simulink library "GTPR_Library"  (R2021a)
settings: Solver=VariableStepAuto  StartTime=0.0  StopTime=10.0  RelTol=1e-3
values from neighbouring files (symbols this model uses):
  aA = 0.5    [SimMechanics_GTPR_OpenLoop_CircularMotion_VS_ClosedLoop.m]
  aB = 0.5    [SimMechanics_GTPR_OpenLoop_CircularMotion_VS_ClosedLoop.m]
  aC = 0.5    [SimMechanics_GTPR_OpenLoop_CircularMotion_VS_ClosedLoop.m]
  alphaAB = deg2rad(120)    [SimMechanics_GTPR_OpenLoop_CircularMotion_VS_ClosedLoop.m]
  alphaAC = deg2rad(240)    [SimMechanics_GTPR_OpenLoop_CircularMotion_VS_ClosedLoop.m]
  eA = 0.28    [SimMechanics_GTPR_OpenLoop_CircularMotion_VS_ClosedLoop.m]
  eB = 0.28    [SimMechanics_GTPR_OpenLoop_CircularMotion_VS_ClosedLoop.m]
  eC = 0.28    [SimMechanics_GTPR_OpenLoop_CircularMotion_VS_ClosedLoop.m]
  g = -9.81    [SimMechanics_GTPR_OpenLoop_CircularMotion_VS_ClosedLoop.m]
  ILA = zeros(3)    [SimMechanics_GTPR_OpenLoop_CircularMotion_VS_ClosedLoop.m]
  IlA = zeros(3)    [SimMechanics_GTPR_OpenLoop_CircularMotion_VS_ClosedLoop.m]
  ILB = zeros(3)    [SimMechanics_GTPR_OpenLoop_CircularMotion_VS_ClosedLoop.m]
  IlB = zeros(3)    [SimMechanics_GTPR_OpenLoop_CircularMotion_VS_ClosedLoop.m]
  ILC = zeros(3)    [SimMechanics_GTPR_OpenLoop_CircularMotion_VS_ClosedLoop.m]
  IlC = zeros(3)    [SimMechanics_GTPR_OpenLoop_CircularMotion_VS_ClosedLoop.m]
  LA = 0.57    [SimMechanics_GTPR_OpenLoop_CircularMotion_VS_ClosedLoop.m]
  lA = 0.9    [SimMechanics_GTPR_OpenLoop_CircularMotion_VS_ClosedLoop.m]
  LB = 0.57    [SimMechanics_GTPR_OpenLoop_CircularMotion_VS_ClosedLoop.m]
  lB = 0.9    [SimMechanics_GTPR_OpenLoop_CircularMotion_VS_ClosedLoop.m]
  LC = 0.57    [SimMechanics_GTPR_OpenLoop_CircularMotion_VS_ClosedLoop.m]
  lC = 0.9    [SimMechanics_GTPR_OpenLoop_CircularMotion_VS_ClosedLoop.m]
  m_unaccounted = 1e-16    [SimMechanics_GTPR_OpenLoop_CircularMotion_VS_ClosedLoop.m]
  mLA = density_upperArm*VLA    (= 1.4415197891)    [SimMechanics_GTPR_OpenLoop_CircularMotion_VS_ClosedLoop.m]
  mlA = density_LowerArm*VlA    (= 0.190851753706)    [SimMechanics_GTPR_OpenLoop_CircularMotion_VS_ClosedLoop.m]
  mLB = density_upperArm*VLB    (= 1.4415197891)    [SimMechanics_GTPR_OpenLoop_CircularMotion_VS_ClosedLoop.m]
  mlB = density_LowerArm*VlB    (= 0.190851753706)    [SimMechanics_GTPR_OpenLoop_CircularMotion_VS_ClosedLoop.m]
  mLC = density_upperArm*VLC    (= 1.4415197891)    [SimMechanics_GTPR_OpenLoop_CircularMotion_VS_ClosedLoop.m]
  mlC = density_LowerArm*VlC    (= 0.190851753706)    [SimMechanics_GTPR_OpenLoop_CircularMotion_VS_ClosedLoop.m]
  mTCP = density_workTriangle * VTCP    [SimMechanics_GTPR_OpenLoop_CircularMotion_VS_ClosedLoop.m]
undefined symbols (not defined in the file or in its folder): dq1, dq2, dq3, q1, q2, q3, X, Y, Z
libraries: sm_lib x83, $bdroot x31, nesl_utility x24
(part 6 of 8)

== matlab function GTPR_Library/Dynamics/DynamicEquations/Dynamic Eqs ==
  data: Mxyz output; Mddq output; aA input size=1; aB input size=1; aC input; alphaAB input size=1; alphaAC input size=1; LA input size=1; LB input size=1; LC input size=1; lA input size=1; lB input size=1; lC input size=1; eA input size=1; eB input size=1; eC input size=1; q input size=[3 1]; dq input size=[3 1]; ddq input size=[3 1]; TCP input size=[3 1]; ILA input size=[3 3]; ILB input size=[3 3]; ILC input size=[3 3]; IlA input size=[3 3]; IlB input size=[3 3]; IlC input size=[3 3]; a input size=[3 1]; g input size=1; mLA input size=1; mLB input size=1; mLC input size=1; mlA input size=1; mlB input size=1; mlC input size=1; mTCP input size=1; dGammasdq output; Fext input size=[3 1]; lambda output; Mtimesddq output; M output; f output; tau output; v input; J11 input; J12 input; J13 input; J21 input; J22 input; J23 input; J31 input; J32 input; J33 input
function [Mxyz, Mddq, dGammasdq, lambda, Mtimesddq, M, f, tau] = Dynamics(aA, aB, aC, alphaAB, alphaAC, LA, LB, LC, lA, lB, lC, eA, eB, eC, q, dq, ddq,TCP, ILA, ILB, ILC, IlA, IlB, IlC, a, g, mLA, mLB, mLC, mlA, mlB, mlC, mTCP, Fext, v, J11, J12, J13, J21, J22, J23, J31, J32, J33) 

alphaAA = 0;

q1 = q(1);
q2 = q(2);
q3 = q(3);

dq1 = dq(1);
dq2 = dq(2);
dq3 = dq(3);

ddq1 = ddq(1);
ddq2 = ddq(2);
ddq3 = ddq(3);

x = TCP(1);
y = TCP(2);
z = TCP(3);

dx = v(1);
dy = v(2);
dz = v(3);

ddx = a(1);
ddy = a(2);
ddz = a(3);

ILAxx = ILA(1,1);
ILAxy = ILA(1,2);
% ILAxz = ILA(1,3);
ILAyy = ILA(2,2);
% ILAyz = ILA(2,3);
% ILAzz = ILA(3,3);

ILBxx = ILB(1,1);
ILBxy = ILB(1,2);
% ILBxz = ILB(1,3);
ILByy = ILB(2,2);
% ILByz = ILB(2,3);
% ILBzz = ILB(3,3);

ILCxx = ILC(1,1);
ILCxy = ILC(1,2);
% ILCxz = ILC(1,3);
ILCyy = ILC(2,2);
% ILCyz = ILC(2,3);
% ILCzz = ILC(3,3);

IlAxx = IlA(1,1);
IlAxy = IlA(1,2);
IlAxz = IlA(1,3);
IlAyy = IlA(2,2);
IlAyz = IlA(2,3);
IlAzz = IlA(3,3);

IlBxx = IlB(1,1);
IlBxy = IlB(1,2);
IlBxz = IlB(1,3);
IlByy = IlB(2,2);
IlByz = IlB(2,3);
IlBzz = IlB(3,3);

IlCxx = IlC(1,1);
IlCxy = IlC(1,2);
IlCxz = IlC(1,3);
IlCyy = IlC(2,2);
IlCyz = IlC(2,3);
IlCzz = IlC(3,3);

J = [J11, J12, J13; J21, J22, J23; J31, J32, J33];

dGammasdxyz = reshape([x.*2.0+aA.*sin(alphaAA).*2.0-eA.*sin(alphaAA).*2.0+LA.*cos(q1).*sin(alphaAA).*2.0,y.*2.0+aA.*cos(alphaAA).*2.0-eA.*cos(alphaAA).*2.0+LA.*cos(alphaAA).*cos(q1).*2.0,z.*2.0+LA.*sin(q1).*2.0,x.*2.0+aB.*sin(alphaAB).*2.0-eB.*sin(alphaAB).*2.0+LB.*cos(q2).*sin(alphaAB).*2.0,y.*2.0+aB.*cos(alphaAB).*2.0-eB.*cos(alphaAB).*2.0+LB.*cos(alphaAB).*cos(q2).*2.0,z.*2.0+LB.*sin(q2).*2.0,x.*2.0+aC.*sin(alphaAC).*2.0-eC.*sin(alphaAC).*2.0+LC.*cos(q3).*sin(alphaAC).*2.0,y.*2.0+aC.*cos(alphaAC).*2.0-eC.*cos(alphaAC).*2.0+LC.*cos(alphaAC).*cos(q3).*2.0,z.*2.0+LC.*sin(q3).*2.0],[3,3]);
Mxyz = [(mlA.*(ddx./2.0+(LA.*dq1.^2.*cos(q1).*cos(alphaAA-pi./2.0))./2.0+(LA.*ddq1.*sin(q1).*cos(alphaAA-pi./2.0))./2.0))./2.0+mlA.*(ddx./4.0+(LA.*dq1.^2.*cos(q1).*cos(alphaAA-pi./2.0))./4.0+(LA.*ddq1.*sin(q1).*cos(alphaAA-pi./2.0))./4.0)+(mlB.*(ddx./2.0+(LB.*dq2.^2.*cos(q2).*cos(alphaAB-pi./2.0))./2.0+(LB.*ddq2.*sin(q2).*cos(alphaAB-pi./2.0))./2.0))./2.0+mlB.*(ddx./4.0+(LB.*dq2.^2.*cos(q2).*cos(alphaAB-pi./2.0))./4.0+(LB.*ddq2.*sin(q2).*cos(alphaAB-pi./2.0))./4.0)+(mlC.*(ddx./2.0+(LC.*dq3.^2.*cos(q3).*cos(alphaAC-pi./2.0))./2.0+(LC.*ddq3.*sin(q3).*cos(alphaAC-pi./2.0))./2.0))./2.0+mlC.*(ddx./4.0+(LC.*dq3.^2.*cos(q3).*cos(alphaAC-pi./2.0))./4.0+(LC.*ddq3.*sin(q3).*cos(alphaAC-pi./2.0))./4.0)+ddx.*mTCP+(((IlAxz.*1.0./lA.^2.*(y+aA.*cos(alphaAA)-eA.*cos(alphaAA)+LA.*cos(alphaAA).*cos(q1)))./2.0-(IlAxy.*1.0./lA.^2.*(z+LA.*sin(q1)))./2.0).*(((dz+LA.*dq1.*cos(q1)).*(dy+LA.*dq1.*sin(alphaAA-pi./2.0).*sin(q1)))./lA-((dy-LA.*dq1.*cos(alphaAA).*sin(q1)).*(dz+LA.*dq1.*sin(pi./2.0).*cos(q1)))./lA+((z+LA.*sin(q1)).*(ddy+LA.*dq1.^2.*sin(alphaAA-pi./2.0).*cos(q1)+LA.*ddq1.*sin(alphaAA-pi./2.0).*sin(q1)))./lA-((ddz+LA.*ddq1.*sin(pi./2.0).*cos(q1)-LA.*dq1.^2.*sin(pi./2.0).*sin(q1)).*(y+aA.*cos(alphaAA)-eA.*cos(alphaAA)+LA.*cos(alphaAA).*cos(q1)))./lA).*2.0)./lA+(((IlBxz.*1.0./lB.^2.*(y+aB.*cos(alphaAB)-eB.*cos(alphaAB)+LB.*cos(alphaAB).*cos(q2)))./2.0-(IlBxy.*1.0./lB.^2.*(z+LB.*sin(q2)))./2.0).*(((dz+LB.*dq2.*cos(q2)).*(dy+LB.*dq2.*sin(alphaAB-pi./2.0).*sin(q2)))./lB-((dy-LB.*dq2.*cos(alphaAB).*sin(q2)).*(dz+LB.*dq2.*sin(pi./2.0).*cos(q2)))./lB+((z+LB.*sin(q2)).*(ddy+LB.*dq2.^2.*sin(alphaAB-pi./2.0).*cos(q2)+LB.*ddq2.*sin(alphaAB-pi./2.0).*sin(q2)))./lB-((ddz+LB.*ddq2.*sin(pi./2.0).*cos(q2)-LB.*dq2.^2.*sin(pi./2.0).*sin(q2)).*(y+aB.*cos(alphaAB)-eB.*cos(alphaAB)+LB.*cos(alphaAB).*cos(q2)))./lB).*2.0)./lB+(((IlCxz.*1.0./lC.^2.*(y+aC.*cos(alphaAC)-eC.*cos(alphaAC)+LC.*cos(alphaAC).*cos(q3)))./2.0-(IlCxy.*1.0./lC.^2.*(z+LC.*sin(q3)))./2.0).*(((dz+LC.*dq3.*cos(q3)).*(dy+LC.*dq3.*sin(alphaAC-pi./2.0).*sin(q3)))./lC-((dy-LC.*dq3.*cos(alphaAC).*sin(q3)).*(dz+LC.*dq3.*sin(pi./2.0).*cos(q3)))./lC+((z+LC.*sin(q3)).*(ddy+LC.*dq3.^2.*sin(alphaAC-pi./2.0).*cos(q3)+LC.*ddq3.*sin(alphaAC-pi./2.0).*sin(q3)))./lC-((ddz+LC.*ddq3.*sin(pi./2.0).*cos(q3)-LC.*dq3.^2.*sin(pi./2.0).*sin(q3)).*(y+aC.*cos(alphaAC)-eC.*cos(alphaAC)+LC.*cos(alphaAC).*cos(q3)))./lC).*2.0)./lC-(((IlAxz.*1.0./lA.^2.*(dy+LA.*dq1.*sin(alphaAA-pi./2.0).*sin(q1)))./2.0-(IlAxy.*1.0./lA.^2.*(dz+LA.*dq1.*sin(pi./2.0).*cos(q1)))./2.0).*(((dz+LA.*dq1.*sin(pi./2.0).*cos(q1)).*(y+aA.*cos(alphaAA)-eA.*cos(alphaAA)+LA.*cos(alphaAA).*cos(q1)))./lA-((z+LA.*sin(q1)).*(dy+LA.*dq1.*sin(alphaAA-pi./2.0).*sin(q1)))./lA).*2.0)./lA-(((IlBxz.*1.0./lB.^2.*(dy+LB.*dq2.*sin(alphaAB-pi./2.0).*sin(q2)))./2.0-(IlBxy.*1.0./lB.^2.*(dz+LB.*dq2.*sin(pi./2.0).*cos(q2)))./2.0).*(((dz+LB.*dq2.*sin(pi./2.0).*cos(q2)).*(y+aB.*cos(alphaAB)-eB.*cos(alphaAB)+LB.*cos(alphaAB).*cos(q2)))./lB-((z+LB.*sin(q2)).*(dy+LB.*dq2.*sin(alphaAB-pi./2.0).*sin(q2)))./lB).*2.0)./lB-(((IlCxz.*1.0./lC.^2.*(dy+LC.*dq3.*sin(alphaAC-pi./2.0).*sin(q3)))./2.0-(IlCxy.*1.0./lC.^2.*(dz+LC.*dq3.*sin(pi./2.0).*cos(q3)))./2.0).*(((dz+LC.*dq3.*sin(pi./2.0).*cos(q3)).*(y+aC.*cos(alphaAC)-eC.*cos(alphaAC)+LC.*cos(alphaAC).*cos(q3)))./lC-((z+LC.*sin(q3)).*(dy+LC.*dq3.*sin(alphaAC-pi./2.0).*sin(q3)))./lC).*2.0)./lC-1.0./lA.^2.*(dy-LA.*dq1.*cos(alphaAA).*sin(q1)).*((IlAzz.*(((dx-LA.*dq1.*sin(q1).*cos(alphaAA-pi./2.0)).*(y+aA.*cos(alphaAA)-eA.*cos(alphaAA)+LA.*cos(alphaAA).*cos(q1)))./lA-((dy+LA.*dq1.*sin(alphaAA-pi./2.0).*sin(q1)).*(x+aA.*sin(alphaAA)-eA.*sin(alphaAA)+LA.*cos(q1).*sin(alphaAA)))./lA).*(-1.0./2.0))./lA+(IlAxz.*(((dz+LA.*dq1.*sin(pi./2.0).*cos(q1)).*(y+aA.*cos(alphaAA)-eA.*cos(alphaAA)+LA.*cos(alphaAA).*cos(q1)))./lA-((z+LA.*sin(q1)).*(dy+LA.*dq1.*sin(alphaAA-pi./2.0).*sin(q1)))./lA))./(lA.*2.0)+(IlAyz.*(((z+LA.*sin(q1)).*(dx-LA.*dq1.*sin(q1).*cos(alphaAA-pi./2.0)))./lA-((dz+LA.*dq1.*sin(pi./2.0).*cos(q1)).*(x+aA.*sin(alphaAA)-eA.*sin(alphaAA)+LA.*cos(q1).*sin(alphaAA)))./lA))./(lA.*2.0)).*2.0-1.0./lB.^2.*(dy-LB.*dq2.*cos(alphaAB).*sin(q2)).*((IlBzz.*(((dx-LB.*dq2.*sin(q2).*cos(alphaAB-pi./2.0)).*(y+aB.*cos(alphaAB)-eB.*cos(alphaAB)+LB.*cos(alphaAB).*cos(q2)))./lB-((dy+LB.*dq2.*sin(alphaAB-pi./2.0).*sin(q2)).*(x+aB.*sin(alphaAB)-eB.*sin(alphaAB)+LB.*cos(q2).*sin(alphaAB)))./lB).*(-1.0./2.0))./lB+(IlBxz.*(((dz+LB.*dq2.*sin(pi./2.0).*cos(q2)).*(y+aB.*cos(alphaAB)-eB.*cos(alphaAB)+LB.*cos(alphaAB).*cos(q2)))./lB-((z+LB.*sin(q2)).*(dy+LB.*dq2.*sin(alphaAB-pi./2.0).*sin(q2)))./lB))./(lB.*2.0)+(IlByz.*(((z+LB.*sin(q2)).*(dx-LB.*dq2.*sin(q2).*cos(alphaAB-pi./2.0)))./lB-((dz+LB.*dq2.*sin(pi./2.0).*cos(q2)).*(x+aB.*sin(alphaAB)-eB.*sin(alphaAB)+LB.*cos(q2).*sin(alphaAB)))./lB))./(lB.*2.0)).*2.0-1.0./lC.^2.*(dy-LC.*dq3.*cos(alphaAC).*sin(q3)).*((IlCzz.*(((dx-LC.*dq3.*sin(q3).*cos(alphaAC-pi./2.0)).*(y+aC.*cos(alphaAC)-eC.*cos(alphaAC)+LC.*cos(alphaAC).*cos(q3)))./lC-((dy+LC.*dq3.*sin(alphaAC-pi./2.0).*sin(q3)).*(x+aC.*sin(alphaAC)-eC.*sin(alphaAC)+LC.*cos(q3).*sin(alphaAC)))./lC).*(-1.0./2.0))./lC+(IlCxz.*(((dz+LC.*dq3.*sin(pi./2.0).*cos(q3)).*(y+aC.*cos(alphaAC)-eC.*cos(alphaAC)+LC.*cos(alphaAC).*cos(q3)))./lC-((z+LC.*sin(q3)).*(dy+LC.*dq3.*sin(alphaAC-pi./2.0).*sin(q3)))./lC))./(lC.*2.0)+(IlCyz.*(((z+LC.*sin(q3)).*(dx-LC.*dq3.*sin(q3).*cos(alphaAC-pi./2.0)))./lC-((dz+LC.*dq3.*sin(pi./2.0).*cos(q3)).*(x+aC.*sin(alphaAC)-eC.*sin(alphaAC)+LC.*cos(q3).*sin(alphaAC)))./lC))./(lC.*2.0)).*2.0-((((z+LA.*sin(q1)).*(dx-LA.*dq1.*sin(q1).*cos(alphaAA-pi./2.0)))./lA-((dz+LA.*dq1.*sin(pi./2.0).*cos(q1)).*(x+aA.*sin(alphaAA)-eA.*sin(alphaAA)+LA.*cos(q1).*sin(alphaAA)))./lA).*((IlAyz.*1.0./lA.^2.*(dy+LA.*dq1.*sin(alphaAA-pi./2.0).*sin(q1)))./2.0-(IlAyy.*1.0./lA.^2.*(dz+LA.*dq1.*sin(pi./2.0).*cos(q1)))./2.0).*2.0)./lA-((((z+LB.*sin(q2)).*(dx-LB.*dq2.*sin(q2).*cos(alphaAB-pi./2.0)))./lB-((dz+LB.*dq2.*sin(pi./2.0).*cos(q2)).*(x+aB.*sin(alphaAB)-eB.*sin(alphaAB)+LB.*cos(q2).*sin(alphaAB)))./lB).*((IlByz.*1.0./lB.^2.*(dy+LB.*dq2.*sin(alphaAB-pi./2.0).*sin(q2)))./2.0-(IlByy.*1.0./lB.^2.*(dz+LB.*dq2.*sin(pi./2.0).*cos(q2)))./2.0).*2.0)./lB-((((z+LC.*sin(q3)).*(dx-LC.*dq3.*sin(q3).*cos(alphaAC-pi./2.0)))./lC-((dz+LC.*dq3.*sin(pi./2.0).*cos(q3)).*(x+aC.*sin(alphaAC)-eC.*sin(alphaAC)+LC.*cos(q3).*sin(alphaAC)))./lC).*((IlCyz.*1.0./lC.^2.*(dy+LC.*dq3.*sin(alphaAC-pi./2.0).*sin(q3)))./2.0-(IlCyy.*1.0./lC.^2.*(dz+LC.*dq3.*sin(pi./2.0).*cos(q3)))./2.0).*2.0)./lC+1.0./lA.^2.*(dz+LA.*dq1.*cos(q1)).*((IlAyz.*(((dx-LA.*dq1.*sin(q1).*cos(alphaAA-pi./2.0)).*(y+aA.*cos(alphaAA)-eA.*cos(alphaAA)+LA.*cos(alphaAA).*cos(q1)))./lA-((dy+LA.*dq1.*sin(alphaAA-pi./2.0).*sin(q1)).*(x+aA.*sin(alphaAA)-eA.*sin(alphaAA)+LA.*cos(q1).*sin(alphaAA)))./lA).*(-1.0./2.0))./lA+(IlAxy.*(((dz+LA.*dq1.*sin(pi./2.0).*cos(q1)).*(y+aA.*cos(alphaAA)-eA.*cos(alphaAA)+LA.*cos(alphaAA).*cos(q1)))./lA-((z+LA.*sin(q1)).*(dy+LA.*dq1.*sin(alphaAA-pi./2.0).*sin(q1)))./lA))./(lA.*2.0)+(IlAyy.*(((z+LA.*sin(q1)).*(dx-LA.*dq1.*sin(q1).*cos(alphaAA-pi./2.0)))./lA-((dz+LA.*dq1.*sin(pi./2.0).*cos(q1)).*(x+aA.*sin(alphaAA)-eA.*sin(alphaAA)+LA.*cos(q1).*sin(alphaAA)))./lA))./(lA.*2.0)).*2.0+1.0./lB.^2.*(dz+LB.*dq2.*cos(q2)).*((IlByz.*(((dx-LB.*dq2.*sin(q2).*cos(alphaAB-pi./2.0)).*(y+aB.*cos(alphaAB)-eB.*cos(alphaAB)+LB.*cos(alphaAB).*cos(q2)))./lB-((dy+LB.*dq2.*sin(alphaAB-pi./2.0).*sin(q2)).*(x+aB.*sin(alphaAB)-eB.*sin(alphaAB)+LB.*cos(q2).*sin(alphaAB)))./lB).*(-1.0./2.0))./lB+(IlBxy.*(((dz+LB.*dq2.*sin(pi./2.0).*cos(q2)).*(y+aB.*cos(alphaAB)-eB.*cos(alphaAB)+LB.*cos(alphaAB).*cos(q2)))./lB-((z+LB.*sin(q2)).*(dy+LB.*dq2.*sin(alphaAB-pi./2.0).*sin(q2)))./lB))./(lB.*2.0)+(IlByy.*(((z+LB.*sin(q2)).*(dx-LB.*dq2.*sin(q2).*cos(alphaAB-pi./2.0)))./lB-((dz+LB.*dq2.*sin(pi./2.0).*cos(q2)).*(x+aB.*sin(alphaAB)-eB.*sin(alphaAB)+LB.*cos(q2).*sin(alphaAB)))./lB))./(lB.*2.0)).*2.0+1.0./lC.^2.*(dz+LC.*dq3.*cos(q3)).*((IlCyz.*(((dx-LC.*dq3.*sin(q3).*cos(alphaAC-pi./2.0)).*(y+aC.*cos(alphaAC)-eC.*cos(alphaAC)+LC.*cos(alphaAC).*cos(q3)))./lC-((dy+LC.*dq3.*sin(alphaAC-pi./2.0).*sin(q3)).*(x+aC.*sin(alphaAC)-eC.*sin(alphaAC)+LC.*cos(q3).*sin(alphaAC)))./lC).*(-1.0./2.0))./lC+(IlCxy.*(((dz+LC.*dq3.*sin(pi./2.0).*cos(q3)).*(y+aC.*cos(alphaAC)-eC.*cos(alphaAC)+LC.*cos(alphaAC).*cos(q3)))./lC-((z+LC.*sin(q3)).*(dy+LC.*dq3.*sin(alphaAC-pi./2.0).*sin(q3)))./lC))./(lC.*2.0)+(IlCyy.*(((z+LC.*sin(q3)).*(dx-LC.*dq3.*sin(q3).*cos(alphaAC-pi./2.0)))./lC-((dz+LC.*dq3.*sin(pi./2.0).*cos(q3)).*(x+aC.*sin(alphaAC)-eC.*sin(alphaAC)+LC.*cos(q3).*sin(alphaAC)))./lC))./(lC.*2.0)).*2.0-(((IlAyz.*1.0./lA.^2.*(dz+LA.*dq1.*cos(q1)))./2.0-(IlAzz.*1.0./lA.^2.*(dy-LA.*dq1.*cos(alphaAA).*sin(q1)))./2.0).*(((dx-LA.*dq1.*sin(q1).*cos(alphaAA-pi./2.0)).*(y+aA.*cos(alphaAA)-eA.*cos(alphaAA)+LA.*cos(alphaAA).*cos(q1)))./lA-((dy+LA.*dq1.*sin(alphaAA-pi./2.0).*sin(q1)).*(x+aA.*sin(alphaAA)-eA.*sin(alphaAA)+LA.*cos(q1).*sin(alphaAA)))./lA).*2.0)./lA-(((IlByz.*1.0./lB.^2.*(dz+LB.*dq2.*cos(q2)))./2.0-(IlBzz.*1.0./lB.^2.*(dy-LB.*dq2.*cos(alphaAB).*sin(q2)))./2.0).*(((dx-LB.*dq2.*sin(q2).*cos(alphaAB-pi./2.0)).*(y+aB.*cos(alphaAB)-eB.*cos(alphaAB)+LB.*cos(alphaAB).*cos(q2)))./lB-((dy+LB.*dq2.*sin(alphaAB-pi./2.0).*sin(q2)).*(x+aB.*sin(alphaAB)-eB.*sin(alphaAB)+LB.*cos(q2).*sin(alphaAB)))./lB).*2.0)./lB-(((IlCyz.*1.0./lC.^2.*(dz+LC.*dq3.*cos(q3)))./2.0-(IlCzz.*1.0./lC.^2.*(dy-LC.*dq3.*cos(alphaAC).*sin(q3)))./2.0).*(((dx-LC.*dq3.*sin(q3).*cos(alphaAC-pi./2.0)).*(y+aC.*cos(alphaAC)-eC.*cos(alphaAC)+LC.*cos(alphaAC).*cos(q3)))./lC-((dy+LC.*dq3.*sin(alphaAC-pi./2.0).*sin(q3)).*(x+aC.*sin(alphaAC)-eC.*sin(alphaAC)+LC.*cos(q3).*sin(alphaAC)))./lC).*2.0)./lC-1.0./lA.^2.*(dy+LA.*dq1.*sin(alphaAA-pi./2.0).*sin(q1)).*((IlAzz.*(((dx-LA.*dq1.*sin(q1).*cos(alphaAA-pi./2.0)).*(y+aA.*cos(alphaAA)-eA.*cos(alphaAA)+LA.*cos(alphaAA).*cos(q1)))./lA-((dy+LA.*dq1.*sin(alphaAA-pi./2.0).*sin(q1)).*(x+aA.*sin(alphaAA)-eA.*sin(alphaAA)+LA.*cos(q1).*sin(alphaAA)))./lA).*(-1.0./2.0))./lA+(IlAxz.*(((dz+LA.*dq1.*sin(pi./2.0).*cos(q1)).*(y+aA.*cos(alphaAA)-eA.*cos(alphaAA)+LA.*cos(alphaAA).*cos(q1)))./lA-((z+LA.*sin(q1)).*(dy+LA.*dq1.*sin(alphaAA-pi./2.0).*sin(q1)))./lA))./(lA.*2.0)+(IlAyz.*(((z+LA.*sin(q1)).*(dx-LA.*dq1.*sin(q1).*cos(alphaAA-pi./2.0)))./lA-((dz+LA.*dq1.*sin(pi./2.0).*cos(q1)).*(x+aA.*sin(alphaAA)-eA.*sin(alphaAA)+LA.*cos(q1).*sin(alphaAA)))./lA))./(lA.*2.0)).*2.0-1.0./lB.^2.*(dy+LB.*dq2.*sin(alphaAB-pi./2.0).*sin(q2)).*((IlBzz.*(((dx-LB.*dq2.*sin(q2).*cos(alphaAB-pi./2.0)).*(y+aB.*cos(alphaAB)-eB.*cos(alphaAB)+LB.*cos(alphaAB).*cos(q2)))./lB-((dy+LB.*dq2.*sin(alphaAB-pi./2.0).*sin(q2)).*(x+aB.*sin(alphaAB)-eB.*sin(alphaAB)+LB.*cos(q2).*sin(alphaAB)))./lB).*(-1.0./2.0))./lB+(IlBxz.*(((dz+LB.*dq2.*sin(pi./2.0).*cos(q2)).*(y+aB.*cos(alphaAB)-eB.*cos(alphaAB)+LB.*cos(alphaAB).*cos(q2)))./lB-((z+LB.*sin(q2)).*(dy+LB.*dq2.*sin(alphaAB-pi./2.0).*sin(q2)))./lB))./(lB.*2.0)+(IlByz.*(((z+LB.*sin(q2)).*(dx-LB.*dq2.*sin(q2).*cos(alphaAB-pi./2.0)))./lB-((dz+LB.*dq2.*sin(pi./2.0).*cos(q2)).*(x+aB.*sin(alphaAB)-eB.*sin(alphaAB)+LB.*cos(q2).*sin(alphaAB)))./lB))./(lB.*2.0)).*2.0-1.0./lC.^2.*(dy+LC.*dq3.*sin(alphaAC-pi./2.0).*sin(q3)).*((IlCzz.*(((dx-LC.*dq3.*sin(q3).*cos(alphaAC-pi./2.0)).*(y+aC.*cos(alphaAC)-eC.*cos(alphaAC)+LC.*cos(alphaAC).*cos(q3)))./lC-((dy+LC.*dq3.*sin(alphaAC-pi./2.0).*sin(q3)).*(x+aC.*sin(alphaAC)-eC.*sin(alphaAC)+LC.*cos(q3).*sin(alphaAC)))./lC).*(-1.0./2.0))./lC+(IlCxz.*(((dz+LC.*dq3.*sin(pi./2.0).*cos(q3)).*(y+aC.*cos(alphaAC)-eC.*cos(alphaAC)+LC.*cos(alphaAC).*cos(q3)))./lC-((z+LC.*sin(q3)).*(dy+LC.*dq3.*sin(alphaAC-pi./2.0).*sin(q3)))./lC))./(lC.*2.0)+(IlCyz.*(((z+LC.*sin(q3)).*(dx-LC.*dq3.*sin(q3).*cos(alphaAC-pi./2.0)))./lC-((dz+LC.*dq3.*sin(pi./2.0).*cos(q3)).*(x+aC.*sin(alphaAC)-eC.*sin(alphaAC)+LC.*cos(q3).*sin(alphaAC)))./lC))./(lC.*2.0)).*2.0-(((IlAzz.*1.0./lA.^2.*(y+aA.*cos(alphaAA)-eA.*cos(alphaAA)+LA.*cos(alphaAA).*cos(q1)))./2.0-(IlAyz.*1.0./lA.^2.*(z+LA.*sin(q1)))./2.0).*(-((dy-LA.*dq1.*cos(alphaAA).*sin(q1)).*(dx-LA.*dq1.*sin(q1).*cos(alphaAA-pi./2.0)))./lA+((dx-LA.*dq1.*sin(alphaAA).*sin(q1)).*(dy+LA.*dq1.*sin(alphaAA-pi./2.0).*sin(q1)))./lA+((ddy+LA.*dq1.^2.*sin(alphaAA-pi./2.0).*cos(q1)+LA.*ddq1.*sin(alphaAA-pi./2.0).*sin(q1)).*(x+aA.*sin(alphaAA)-eA.*sin(alphaAA)+LA.*cos(q1).*sin(alphaAA)))./lA+((-ddx+LA.*dq1.^2.*cos(q1).*cos(alphaAA-pi./2.0)+LA.*ddq1.*sin(q1).*cos(alphaAA-pi./2.0)).*(y+aA.*cos(alphaAA)-eA.*cos(alphaAA)+LA.*cos(alphaAA).*cos(q1)))./lA).*2.0)./lA-(((IlBzz.*1.0./lB.^2.*(y+aB.*cos(alphaAB)-eB.*cos(alphaAB)+LB.*cos(alphaAB).*cos(q2)))./2.0-(IlByz.*1.0./lB.^2.*(z+LB.*sin(q2)))./2.0).*(-((dy-LB.*dq2.*cos(alphaAB).*sin(q2)).*(dx-LB.*dq2.*sin(q2).*cos(alphaAB-pi./2.0)))./lB+((dx-LB.*dq2.*sin(alphaAB).*sin(q2)).*(dy+LB.*dq2.*sin(alphaAB-pi./2.0).*sin(q2)))./lB+((ddy+LB.*dq2.^2.*sin(alphaAB-pi./2.0).*cos(q2)+LB.*ddq2.*sin(alphaAB-pi./2.0).*sin(q2)).*(x+aB.*sin(alphaAB)-eB.*sin(alphaAB)+LB.*cos(q2).*sin(alphaAB)))./lB+((-ddx+LB.*dq2.^2.*cos(q2).*cos(alphaAB-pi./2.0)+LB.*ddq2.*sin(q2).*cos(alphaAB-pi./2.0)).*(y+aB.*cos(alphaAB)-eB.*cos(alphaAB)+LB.*cos(alphaAB).*cos(q2)))./lB).*2.0)./lB-(((IlCzz.*1.0./lC.^2.*(y+aC.*cos(alphaAC)-eC.*cos(alphaAC)+LC.*cos(alphaAC).*cos(q3)))./2.0-(IlCyz.*1.0./lC.^2.*(z+LC.*sin(q3)))./2.0).*(-((dy-LC.*dq3.*cos(alphaAC).*sin(q3)).*(dx-LC.*dq3.*sin(q3).*cos(alphaAC-pi./2.0)))./lC+((dx-LC.*dq3.*sin(alphaAC).*sin(q3)).*(dy+LC.*dq3.*sin(alphaAC-pi./2.0).*sin(q3)))./lC+((ddy+LC.*dq3.^2.*sin(alphaAC-pi./2.0).*cos(q3)+LC.*ddq3.*sin(alphaAC-pi./2.0).*sin(q3)).*(x+aC.*sin(alphaAC)-eC.*sin(alphaAC)+LC.*cos(q3).*sin(alphaAC)))./lC+((-ddx+LC.*dq3.^2.*cos(q3).*cos(alphaAC-pi./2.0)+LC.*ddq3.*sin(q3).*cos(alphaAC-pi./2.0)).*(y+aC.*cos(alphaAC)-eC.*cos(alphaAC)+LC.*cos(alphaAC).*cos(q3)))./lC).*2.0)./lC+(((IlAyz.*1.0./lA.^2.*(y+aA.*cos(alphaAA)-eA.*cos(alphaAA)+LA.*cos(alphaAA).*cos(q1)))./2.0-(IlAyy.*1.0./lA.^2.*(z+LA.*sin(q1)))./2.0).*(((ddz+LA.*ddq1.*sin(pi./2.0).*cos(q1)-LA.*dq1.^2.*sin(pi./2.0).*sin(q1)).*(x+aA.*sin(alphaAA)-eA.*sin(alphaAA)+LA.*cos(q1).*sin(alphaAA)))./lA-((dz+LA.*dq1.*cos(q1)).*(dx-LA.*dq1.*sin(q1).*cos(alphaAA-pi./2.0)))./lA+((dx-LA.*dq1.*sin(alphaAA).*sin(q1)).*(dz+LA.*dq1.*sin(pi./2.0).*cos(q1)))./lA+((z+LA.*sin(q1)).*(-ddx+LA.*dq1.^2.*cos(q1).*cos(alphaAA-pi./2.0)+LA.*ddq1.*sin(q1).*cos(alphaAA-pi./2.0)))./lA).*2.0)./lA+(((IlByz.*1.0./lB.^2.*(y+aB.*cos(alphaAB)-eB.*cos(alphaAB)+LB.*cos(alphaAB).*cos(q2)))./2.0-(IlByy.*1.0./lB.^2.*(z+LB.*sin(q2)))./2.0).*(((ddz+LB.*ddq2.*sin(pi./2.0).*cos(q2)-LB.*dq2.^2.*sin(pi./2.0).*sin(q2)).*(x+aB.*sin(alphaAB)-eB.*sin(alphaAB)+LB.*cos(q2).*sin(alphaAB)))./lB-((dz+LB.*dq2.*cos(q2)).*(dx-LB.*dq2.*sin(q2).*cos(alphaAB-pi./2.0)))./lB+((dx-LB.*dq2.*sin(alphaAB).*sin(q2)).*(dz+LB.*dq2.*sin(pi./2.0).*cos(q2)))./lB+((z+LB.*sin(q2)).*(-ddx+LB.*dq2.^2.*cos(q2).*cos(alphaAB-pi./2.0)+LB.*ddq2.*sin(q2).*cos(alphaAB-pi./2.0)))./lB).*2.0)./lB+(((IlCyz.*1.0./lC.^2.*(y+aC.*cos(alphaAC)-eC.*cos(alphaAC)+LC.*cos(alphaAC).*cos(q3)))./2.0-(IlCyy.*1.0./lC.^2.*(z+LC.*sin(q3)))./2.0).*(((ddz+LC.*ddq3.*sin(pi./2.0).*cos(q3)-LC.*dq3.^2.*sin(pi./2.0).*sin(q3)).*(x+aC.*sin(alphaAC)-eC.*sin(alphaAC)+LC.*cos(q3).*sin(alphaAC)))./lC-((dz+LC.*dq3.*cos(q3)).*(dx-LC.*dq3.*sin(q3).*cos(alphaAC-pi./2.0)))./lC+((dx-LC.*dq3.*sin(alphaAC).*sin(q3)).*(dz+LC.*dq3.*sin(pi./2.0).*cos(q3)))./lC+((z+LC.*sin(q3)).*(-ddx+LC.*dq3.^2.*cos(q3).*cos(alphaAC-pi./2.0)+LC.*ddq3.*sin(q3).*cos(alphaAC-pi./2.0)))./lC).*2.0)./lC+1.0./lA.^2.*(dz+LA.*dq1.*sin(pi./2.0).*cos(q1)).*((IlAyz.*(((dx-LA.*dq1.*sin(q1).*cos(alphaAA-pi./2.0)).*(y+aA.*cos(alphaAA)-eA.*cos(alphaAA)+LA.*cos(alphaAA).*cos(q1)))./lA-((dy+LA.*dq1.*sin(alphaAA-pi./2.0).*sin(q1)).*(x+aA.*sin(alphaAA)-eA.*sin(alphaAA)+LA.*cos(q1).*sin(alphaAA)))./lA).*(-1.0./2.0))./lA+(IlAxy.*(((dz+LA.*dq1.*sin(pi./2.0).*cos(q1)).*(y+aA.*cos(alphaAA)-eA.*cos(alphaAA)+LA.*cos(alphaAA).*cos(q1)))./lA-((z+LA.*sin(q1)).*(dy+LA.*dq1.*sin(alphaAA-pi./2.0).*sin(q1)))./lA))./(lA.*2.0)+(IlAyy.*(((z+LA.*sin(q1)).*(dx-LA.*dq1.*sin(q1).*cos(alphaAA-pi./2.0)))./lA-((dz+LA.*dq1.*sin(pi./2.0).*cos(q1)).*(x+aA.*sin(alphaAA)-eA.*sin(alphaAA)+LA.*cos(q1).*sin(alphaAA)))./lA))./(lA.*2.0)).*2.0+1.0./lB.^2.*(dz+LB.*dq2.*sin(pi./2.0).*cos(q2)).*((IlByz.*(((dx-LB.*dq2.*sin(q2).*cos(alphaAB-pi./2.0)).*(y+aB.*cos(alphaAB)-eB.*cos(alphaAB)+LB.*cos(alphaAB).*cos(q2)))./lB-((dy+LB.*dq2.*sin(alphaAB-pi./2.0).*sin(q2)).*(x+aB.*sin(alphaAB)-eB.*sin(alphaAB)+LB.*cos(q2).*sin(alphaAB)))./lB).*(-1.0./2.0))./lB+(IlBxy.*(((dz+LB.*dq2.*sin(pi./2.0).*cos(q2)).*(y+aB.*cos(alphaAB)-eB.*cos(alphaAB)+LB.*cos(alphaAB).*cos(q2)))./lB-((z+LB.*sin(q2)).*(dy+LB.*dq2.*sin(alphaAB-pi./2.0).*sin(q2)))./lB))./(lB.*2.0)+(IlByy.*(((z+LB.*sin(q2)).*(dx-LB.*dq2.*sin(q2).*cos(alphaAB-pi./2.0)))./lB-((dz+LB.*dq2.*sin(pi./2.0).*cos(q2)).*(x+aB.*sin(alphaAB)-eB.*sin(alphaAB)+LB.*cos(q2).*sin(alphaAB)))./lB))./(lB.*2.0)).*2.0+1.0./lC.^2.*(dz+LC.*dq3.*sin(pi./2.0).*cos(q3)).*((IlCyz.*(((dx-LC.*dq3.*sin(q3).*cos(alphaAC-pi./2.0)).*(y+aC.*cos(alphaAC)-eC.*cos(alphaAC)+LC.*cos(alphaAC).*cos(q3)))./lC-((dy+LC.*dq3.*sin(alphaAC-pi./2.0).*sin(q3)).*(x+aC.*sin(alphaAC)-eC.*sin(alphaAC)+LC.*cos(q3).*sin(alphaAC)))./lC).*(-1.0./2.0))./lC+(IlCxy.*(((dz+LC.*dq3.*sin(pi./2.0).*cos(q3)).*(y+aC.*cos(alphaAC)-eC.*cos(alphaAC)+LC.*cos(alphaAC).*cos(q3)))./lC-((z+LC.*sin(q3)).*(dy+LC.*dq3.*sin(alphaAC-pi./2.0).*sin(q3)))./lC))./(lC.*2.0)+(IlCyy.*(((z+LC.*sin(q3)).*(dx-LC.*dq3.*sin(q3).*cos(alphaAC-pi./2.0)))./lC-((dz+LC.*dq3.*sin(pi./2.0).*cos(q3)).*(x+aC.*sin(alphaAC)-eC.*sin(alphaAC)+LC.*cos(q3).*sin(alphaAC)))./lC))./(lC.*2.0)).*2.0+(((IlAxy.*1.0./lA.^2.*(dz+LA.*dq1.*cos(q1)))./2.0-(IlAxz.*1.0./lA.^2.*(dy-LA.*dq1.*cos(alphaAA).*sin(q1)))./2.0).*(((dz+LA.*dq1.*sin(pi./2.0).*cos(q1)).*(y+aA.*cos(alphaAA)-eA.*cos(alphaAA)+LA.*cos(alphaAA).*cos(q1)))./lA-((z+LA.*sin(q1)).*(dy+LA.*dq1.*sin(alphaAA-pi./2.0).*sin(q1)))./lA).*2.0)./lA+(((IlBxy.*1.0./lB.^2.*(dz+LB.*dq2.*cos(q2)))./2.0-(IlBxz.*1.0./lB.^2.*(dy-LB.*dq2.*cos(alphaAB).*sin(q2)))./2.0).*(((dz+LB.*dq2.*sin(pi./2.0).*cos(q2)).*(y+aB.*cos(alphaAB)-eB.*cos(alphaAB)+LB.*cos(alphaAB).*cos(q2)))./lB-((z+LB.*sin(q2)).*(dy+LB.*dq2.*sin(alphaAB-pi./2.0).*sin(q2)))./lB).*2.0)./lB+(((IlCxy.*1.0./lC.^2.*(dz+LC.*dq3.*cos(q3)))./2.0-(IlCxz.*1.0./lC.^2.*(dy-LC.*dq3.*cos(alphaAC).*sin(q3)))./2.0).*(((dz+LC.*dq3.*sin(pi./2.0).*cos(q3)).*(y+aC.*cos(alphaAC)-eC.*cos(alphaAC)+LC.*cos(alphaAC).*cos(q3)))./lC-((z+LC.*sin(q3)).*(dy+LC.*dq3.*sin(alphaAC-pi./2.0).*sin(q3)))./lC).*2.0)./lC+((((z+LA.*sin(q1)).*(dx-LA.*dq1.*sin(q1).*cos(alphaAA-pi./2.0)))./lA-((dz+LA.*dq1.*sin(pi./2.0).*cos(q1)).*(x+aA.*sin(alphaAA)-eA.*sin(alphaAA)+LA.*cos(q1).*sin(alphaAA)))./lA).*((IlAyy.*1.0./lA.^2.*(dz+LA.*dq1.*cos(q1)))./2.0-(IlAyz.*1.0./lA.^2.*(dy-LA.*dq1.*cos(alphaAA).*sin(q1)))./2.0).*2.0)./lA+((((z+LB.*sin(q2)).*(dx-LB.*dq2.*sin(q2).*cos(alphaAB-pi./2.0)))./lB-((dz+LB.*dq2.*sin(pi./2.0).*cos(q2)).*(x+aB.*sin(alphaAB)-eB.*sin(alphaAB)+LB.*cos(q2).*sin(alphaAB)))./lB).*((IlByy.*1.0./lB.^2.*(dz+LB.*dq2.*cos(q2)))./2.0-(IlByz.*1.0./lB.^2.*(dy-LB.*dq2.*cos(alphaAB).*sin(q2)))./2.0).*2.0)./lB+((((z+LC.*sin(q3)).*(dx-LC.*dq3.*sin(q3).*cos(alphaAC-pi./2.0)))./lC-((dz+LC.*dq3.*sin(pi./2.0).*cos(q3)).*(x+aC.*sin(alphaAC)-eC.*sin(alphaAC)+LC.*cos(q3).*sin(alphaAC)))./lC).*((IlCyy.*1.0./lC.^2.*(dz+LC.*dq3.*cos(q3)))./2.0-(IlCyz.*1.0./lC.^2.*(dy-LC.*dq3.*cos(alphaAC).*sin(q3)))./2.0).*2.0)./lC+1.0./lA.^2.*((IlAxz.*(((dz+LA.*dq1.*cos(q1)).*(dy+LA.*dq1.*sin(alphaAA-pi./2.0).*sin(q1)))./lA-((dy-LA.*dq1.*cos(alphaAA).*sin(q1)).*(dz+LA.*dq1.*sin(pi./2.0).*cos(q1)))./lA+((z+LA.*sin(q1)).*(ddy+LA.*dq1.^2.*sin(alphaAA-pi./2.0).*cos(q1)+LA.*ddq1.*sin(alphaAA-pi./2.0).*sin(q1)))./lA-((ddz+LA.*ddq1.*sin(pi./2.0).*cos(q1)-LA.*dq1.^2.*sin(pi./2.0).*sin(q1)).*(y+aA.*cos(alphaAA)-eA.*cos(alphaAA)+LA.*cos(alphaAA).*cos(q1)))./lA))./(lA.*2.0)-(IlAzz.*(-((dy-LA.*dq1.*cos(alphaAA).*sin(q1)).*(dx-LA.*dq1.*sin(q1).*cos(alphaAA-pi./2.0)))./lA+((dx-LA.*dq1.*sin(alphaAA).*sin(q1)).*(dy+LA.*dq1.*sin(alphaAA-pi./2.0).*sin(q1)))./lA+((ddy+LA.*dq1.^2.*sin(alphaAA-pi./2.0).*cos(q1)+LA.*ddq1.*sin(alphaAA-pi./2.0).*sin(q1)).*(x+aA.*sin(alphaAA)-eA.*sin(alphaAA)+LA.*cos(q1).*sin(alphaAA)))./lA+((-ddx+LA.*dq1.^2.*cos(q1).*cos(alphaAA-pi./2.0)+LA.*ddq1.*sin(q1).*cos(alphaAA-pi./2.0)).*(y+aA.*cos(alphaAA)-eA.*cos(alphaAA)+LA.*cos(alphaAA).*cos(q1)))./lA))./(lA.*2.0)+(IlAyz.*(((ddz+LA.*ddq1.*sin(pi./2.0).*cos(q1)-LA.*dq1.^2.*sin(pi./2.0).*sin(q1)).*(x+aA.*sin(alphaAA)-eA.*sin(alphaAA)+LA.*cos(q1).*sin(alphaAA)))./lA-((dz+LA.*dq1.*cos(q1)).*(dx-LA.*dq1.*sin(q1).*cos(alphaAA-pi./2.0)))./lA+((dx-LA.*dq1.*sin(alphaAA).*sin(q1)).*(dz+LA.*dq1.*sin(pi./2.0).*cos(q1)))./lA+((z+LA.*sin(q1)).*(-ddx+LA.*dq1.^2.*cos(q1).*cos(alphaAA-pi./2.0)+LA.*ddq1.*sin(q1).*cos(alphaAA-pi./2.0)))./lA))./(lA.*2.0)).*(y+aA.*cos(alphaAA)-eA.*cos(alphaAA)+LA.*cos(alphaAA).*cos(q1)).*2.0+1.0./lB.^2.*((IlBxz.*(((dz+LB.*dq2.*cos(q2)).*(dy+LB.*dq2.*sin(alphaAB-pi./2.0).*sin(q2)))./lB-((dy-LB.*dq2.*cos(alphaAB).*sin(q2)).*(dz+LB.*dq2.*sin(pi./2.0).*cos(q2)))./lB+((z+LB.*sin(q2)).*(ddy+LB.*dq2.^2.*sin(alphaAB-pi./2.0).*cos(q2)+LB.*ddq2.*sin(alphaAB-pi./2.0).*sin(q2)))./lB-((ddz+LB.*ddq2.*sin(pi./2.0).*cos(q2)-LB.*dq2.^2.*sin(pi./2.0).*sin(q2)).*(y+aB.*cos(alphaAB)-eB.*cos(alphaAB)+LB.*cos(alphaAB).*cos(q2)))./lB))./(lB.*2.0)-(IlBzz.*(-((dy-LB.*dq2.*cos(alphaAB).*sin(q2)).*(dx-LB.*dq2.*sin(q2).*cos(alphaAB-pi./2.0)))./lB+((dx-LB.*dq2.*sin(alphaAB).*sin(q2)).*(dy+LB.*dq2.*sin(alphaAB-pi./2.0).*sin(q2)))./lB+((ddy+LB.*dq2.^2.*sin(alphaAB-pi./2.0).*cos(q2)+LB.*ddq2.*sin(alphaAB-pi./2.0).*sin(q2)).*(x+aB.*sin(alphaAB)-eB.*sin(alphaAB)+LB.*cos(q2).*sin(alphaAB)))./lB+((-ddx+LB.*dq2.^2.*cos(q2).*cos(alphaAB-pi./2.0)+LB.*ddq2.*sin(q2).*cos(alphaAB-pi./2.0)).*(y+aB.*cos(alphaAB)-eB.*cos(alphaAB)+LB.*cos(alphaAB).*cos(q2)))./lB))./(lB.*2.0)+(IlByz.*(((ddz+LB.*ddq2.*sin(pi./2.0).*cos(q2)-LB.*dq2.^2.*sin(pi./2.0).*sin(q2)).*(x+aB.*sin(alphaAB)-eB.*sin(alphaAB)+LB.*cos(q2).*sin(alphaAB)))./lB-((dz+LB.*dq2.*cos(q2)).*(dx-LB.*dq2.*sin(q2).*cos(alphaAB-pi./2.0)))./lB+((dx-LB.*dq2.*sin(alphaAB).*sin(q2)).*(dz+LB.*dq2.*sin(pi./2.0).*cos(q2)))./lB+((z+LB.*sin(q2)).*(-ddx+LB.*dq2.^2.*cos(q2).*cos(alphaAB-pi./2.0)+LB.*ddq2.*sin(q2).*cos(alphaAB-pi./2.0)))./lB))./(lB.*2.0)).*(y+aB.*cos(alphaAB)-eB.*cos(alphaAB)+LB.*cos(alphaAB).*cos(q2)).*2.0+1.0./lC.^2.*((IlCxz.*(((dz+LC.*dq3.*cos(q3)).*(dy+LC.*dq3.*sin(alphaAC-pi./2.0).*sin(q3)))./lC-((dy-LC.*dq3.*cos(alphaAC).*sin(q3)).*(dz+LC.*dq3.*sin(pi./2.0).*cos(q3)))./lC+((z+LC.*sin(q3)).*(ddy+LC.*dq3.^2.*sin(alphaAC-pi./2.0).*cos(q3)+LC.*ddq3.*sin(alphaAC-pi./2.0).*sin(q3)))./lC-((ddz+LC.*ddq3.*sin(pi./2.0).*cos(q3)-LC.*dq3.^2.*sin(pi./2.0).*sin(q3)).*(y+aC.*cos(alphaAC)-eC.*cos(alphaAC)+LC.*cos(alphaAC).*cos(q3)))./lC))./(lC.*2.0)-(IlCzz.*(-((dy-LC.*dq3.*cos(alphaAC).*sin(q3)).*(dx-LC.*dq3.*sin(q3).*cos(alphaAC-pi./2.0)))./lC+((dx-LC.*dq3.*sin(alphaAC).*sin(q3)).*(dy+LC.*dq3.*sin(alphaAC-pi./2.0).*sin(q3)))./lC+((ddy+LC.*dq3.^2.*sin(alphaAC-pi./2.0).*cos(q3)+LC.*ddq3.*sin(alphaAC-pi./2.0).*sin(q3)).*(x+aC.*sin(alphaAC)-eC.*sin(alphaAC)+LC.*cos(q3).*sin(alphaAC)))./lC+((-ddx+LC.*dq3.^2.*cos(q3).*cos(alphaAC-pi./2.0)+LC.*ddq3.*sin(q3).*cos(alphaAC-pi./2.0)).*(y+aC.*cos(alphaAC)-eC.*cos(alphaAC)+LC.*cos(alphaAC).*cos(q3)))./lC))./(lC.*2.0)+(IlCyz.*(((ddz+LC.*ddq3.*sin(pi./2.0).*cos(q3)-LC.*dq3.^2.*sin(pi./2.0).*sin(q3)).*(x+aC.*sin(alphaAC)-eC.*sin(alphaAC)+LC.*cos(q3).*sin(alphaAC)))./lC-((dz+LC.*dq3.*cos(q3)).*(dx-LC.*dq3.*sin(q3).*cos(alphaAC-pi./2.0)))./lC+((dx-LC.*dq3.*sin(alphaAC).*sin(q3)).*(dz+LC.*dq3.*sin(pi./2.0).*cos(q3)))./lC+((z+LC.*sin(q3)).*(-ddx+LC.*dq3.^2.*cos(q3).*cos(alphaAC-pi./2.0)+LC.*ddq3.*sin(q3).*cos(alphaAC-pi./2.0)))./lC))./(lC.*2.0)).*(y+aC.*cos(alphaAC)-eC.*cos(alphaAC)+LC.*cos(alphaAC).*cos(q3)).*2.0+((((dx-LA.*dq1.*sin(q1).*cos(alphaAA-pi./2.0)).*(y+aA.*cos(alphaAA)-eA.*cos(alphaAA)+LA.*cos(alphaAA).*cos(q1)))./lA-((dy+LA.*dq1.*sin(alphaAA-pi./2.0).*sin(q1)).*(x+aA.*sin(alphaAA)-eA.*sin(alphaAA)+LA.*cos(q1).*sin(alphaAA)))./lA).*((IlAzz.*1.0./lA.^2.*(dy+LA.*dq1.*sin(alphaAA-pi./2.0).*sin(q1)))./2.0-(IlAyz.*1.0./lA.^2.*(dz+LA.*dq1.*sin(pi./2.0).*cos(q1)))./2.0).*2.0)./lA+((((dx-LB.*dq2.*sin(q2).*cos(alphaAB-pi./2.0)).*(y+aB.*cos(alphaAB)-eB.*cos(alphaAB)+LB.*cos(alphaAB).*cos(q2)))./lB-((dy+LB.*dq2.*sin(alphaAB-pi./2.0).*sin(q2)).*(x+aB.*sin(alphaAB)-eB.*sin(alphaAB)+LB.*cos(q2).*sin(alphaAB)))./lB).*((IlBzz.*1.0./lB.^2.*(dy+LB.*dq2.*sin(alphaAB-pi./2.0).*sin(q2)))./2.0-(IlByz.*1.0./lB.^2.*(dz+LB.*dq2.*sin(pi./2.0).*cos(q2)))./2.0).*2.0)./lB+((((dx-LC.*dq3.*sin(q3).*cos(alphaAC-pi./2.0)).*(y+aC.*cos(alphaAC)-eC.*cos(alphaAC)+LC.*cos(alphaAC).*cos(q3)))./lC-((dy+LC.*dq3.*sin(alphaAC-pi./2.0).*sin(q3)).*(x+aC.*sin(alphaAC)-eC.*sin(alphaAC)+LC.*cos(q3).*sin(alphaAC)))./lC).*((IlCzz.*1.0./lC.^2.*(dy+LC.*dq3.*sin(alphaAC-pi./2.0).*sin(q3)))./2.0-(IlCyz.*1.0./lC.^2.*(dz+LC.*dq3.*sin(pi./2.0).*cos(q3)))./2.0).*2.0)./lC-1.0./lA.^2.*(z+LA.*sin(q1)).*((IlAxy.*(((dz+LA.*dq1.*cos(q1)).*(dy+LA.*dq1.*sin(alphaAA-pi./2.0).*sin(q1)))./lA-((dy-LA.*dq1.*cos(alphaAA).*sin(q1)).*(dz+LA.*dq1.*sin(pi./2.0).*cos(q1)))./lA+((z+LA.*sin(q1)).*(ddy+LA.*dq1.^2.*sin(alphaAA-pi./2.0).*cos(q1)+LA.*ddq1.*sin(alphaAA-pi./2.0).*sin(q1)))./lA-((ddz+LA.*ddq1.*sin(pi./2.0).*cos(q1)-LA.*dq1.^2.*sin(pi./2.0).*sin(q1)).*(y+aA.*cos(alphaAA)-eA.*cos(alphaAA)+LA.*cos(alphaAA).*cos(q1)))./lA))./(lA.*2.0)-(IlAyz.*(-((dy-LA.*dq1.*cos(alphaAA).*sin(q1)).*(dx-LA.*dq1.*sin(q1).*cos(alphaAA-pi./2.0)))./lA+((dx-LA.*dq1.*sin(alphaAA).*sin(q1)).*(dy+LA.*dq1.*sin(alphaAA-pi./2.0).*sin(q1)))./lA+((ddy+LA.*dq1.^2.*sin(alphaAA-pi./2.0).*cos(q1)+LA.*ddq1.*sin(alphaAA-pi./2.0).*sin(q1)).*(x+aA.*sin(alphaAA)-eA.*sin(alphaAA)+LA.*cos(q1).*sin(alphaAA)))./lA+((-ddx+LA.*dq1.^2.*cos(q1).*cos(alphaAA-pi./2.0)+LA.*ddq1.*sin(q1).*cos(alphaAA-pi./2.0)).*(y+aA.*cos(alphaAA)-eA.*cos(alphaAA)+LA.*cos(alphaAA).*cos(q1)))./lA))./(lA.*2.0)+(IlAyy.*(((ddz+LA.*ddq1.*sin(pi./2.0).*cos(q1)-LA.*dq1.^2.*sin(pi./2.0).*sin(q1)).*(x+aA.*sin(alphaAA)-eA.*sin(alphaAA)+LA.*cos(q1).*sin(alphaAA)))./lA-((dz+LA.*dq1.*cos(q1)).*(dx-LA.*dq1.*sin(q1).*cos(alphaAA-pi./2.0)))./lA+((dx-LA.*dq1.*sin(alphaAA).*sin(q1)).*(dz+LA.*dq1.*sin(pi./2.0).*cos(q1)))./lA+((z+LA.*sin(q1)).*(-ddx+LA.*dq1.^2.*cos(q1).*cos(alphaAA-pi./2.0)+LA.*ddq1.*sin(q1).*cos(alphaAA-pi./2.0)))./lA))./(lA.*2.0)).*2.0-1.0./lB.^2.*(z+LB.*sin(q2)).*((IlBxy.*(((dz+LB.*dq2.*cos(q2)).*(dy+LB.*dq2.*sin(alphaAB-pi./2.0).*sin(q2)))./lB-((dy-LB.*dq2.*cos(alphaAB).*sin(q2)).*(dz+LB.*dq2.*sin(pi./2.0).*cos(q2)))./lB+((z+LB.*sin(q2)).*(ddy+LB.*dq2.^2.*sin(alphaAB-pi./2.0).*cos(q2)+LB.*ddq2.*sin(alphaAB-pi./2.0).*sin(q2)))./lB-((ddz+LB.*ddq2.*sin(pi./2.0).*cos(q2)-LB.*dq2.^2.*sin(pi./2.0).*sin(q2)).*(y+aB.*cos(alphaAB)-eB.*cos(alphaAB)+LB.*cos(alphaAB).*cos(q2)))./lB))./(lB.*2.0)-(IlByz.*(-((dy-LB.*dq2.*cos(alphaAB).*sin(q2)).*(dx-LB.*dq2.*sin(q2).*cos(alphaAB-pi./2.0)))./lB+((dx-LB.*dq2.*sin(alphaAB).*sin(q2)).*(dy+LB.*dq2.*sin(alphaAB-pi./2.0).*sin(q2)))./lB+((ddy+LB.*dq2.^2.*sin(alphaAB-pi./2.0).*cos(q2)+LB.*ddq2.*sin(alphaAB-pi./2.0).*sin(q2)).*(x+aB.*sin(alphaAB)-eB.*sin(alphaAB)+LB.*cos(q2).*sin(alphaAB)))./lB+((-ddx+LB.*dq2.^2.*cos(q2).*cos(alphaAB-pi./2.0)+LB.*ddq2.*sin(q2).*cos(alphaAB-pi./2.0)).*(y+aB.*cos(alphaAB)-eB.*cos(alphaAB)+LB.*cos(alphaAB).*cos(q2)))./lB))./(lB.*2.0)+(IlByy.*(((ddz+LB.*ddq2.*sin(pi./2.0).*cos(q2)-LB.*dq2.^2.*sin(pi./2.0).*sin(q2)).*(x+aB.*sin(alphaAB)-eB.*sin(alphaAB)+LB.*cos(q2).*sin(alphaAB)))./lB-((dz+LB.*dq2.*cos(q2)).*(dx-LB.*dq2.*sin(q2).*cos(alphaAB-pi./2.0)))./lB+((dx-LB.*dq2.*sin(alphaAB).*sin(q2)).*(dz+LB.*dq2.*sin(pi./2.0).*cos(q2)))./lB+((z+LB.*sin(q2)).*(-ddx+LB.*dq2.^2.*cos(q2).*cos(alphaAB-pi./2.0)+LB.*ddq2.*sin(q2).*cos(alphaAB-pi./2.0)))./lB))./(lB.*2.0)).*2.0-1.0./lC.^2.*(z+LC.*sin(q3)).*((IlCxy.*(((dz+LC.*dq3.*cos(q3)).*(dy+LC.*dq3.*sin(alphaAC-pi./2.0).*sin(q3)))./lC-((dy-LC.*dq3.*cos(alphaAC).*sin(q3)).*(dz+LC.*dq3.*sin(pi./2.0).*cos(q3)))./lC+((z+LC.*sin(q3)).*(ddy+LC.*dq3.^2.*sin(alphaAC-pi./2.0).*cos(q3)+LC.*ddq3.*sin(alphaAC-pi./2.0).*sin(q3)))./lC-((ddz+LC.*ddq3.*sin(pi./2.0).*cos(q3)-LC.*dq3.^2.*sin(pi./2.0).*sin(q3)).*(y+aC.*cos(alphaAC)-eC.*cos(alphaAC)+LC.*cos(alphaAC).*cos(q3)))./lC))./(lC.*2.0)-(IlCyz.*(-((dy-LC.*dq3.*cos(alphaAC).*sin(q3)).*(dx-LC.*dq3.*sin(q3).*cos(alphaAC-pi./2.0)))./lC+((dx-LC.*dq3.*sin(alphaAC).*sin(q3)).*(dy+LC.*dq3.*sin(alphaAC-pi./2.0).*sin(q3)))./lC+((ddy+LC.*dq3.^2.*sin(alphaAC-pi./2.0).*cos(q3)+LC.*ddq3.*sin(alphaAC-pi./2.0).*sin(q3)).*(x+aC.*sin(alphaAC)-eC.*sin(alphaAC)+LC.*cos(q3).*sin(alphaAC)))./lC+((-ddx+LC.*dq3.^2.*cos(q3).*cos(alphaAC-pi./2.0)+LC.*ddq3.*sin(q3).*cos(alphaAC-pi./2.0)).*(y+aC.*cos(alphaAC)-eC.*cos(alphaAC)+LC.*cos(alphaAC).*cos(q3)))./lC))./(lC.*2.0)+(IlCyy.*(((ddz+LC.*ddq3.*sin(pi./2.0).*cos(q3)-LC.*dq3.^2.*sin(pi./2.0).*sin(q3)).*(x+aC.*sin(alphaAC)-eC.*sin(alphaAC)+LC.*cos(q3).*sin(alphaAC)))./lC-((dz+LC.*dq3.*cos(q3)).*(dx-LC.*dq3.*sin(q3).*cos(alphaAC-pi./2.0)))./lC+((dx-LC.*dq3.*sin(alphaAC).*sin(q3)).*(dz+LC.*dq3.*sin(pi./2.0).*cos(q3)))./lC+((z+LC.*sin(q3)).*(-ddx+LC.*dq3.^2.*cos(q3).*cos(alphaAC-pi./2.0)+LC.*ddq3.*sin(q3).*cos(alphaAC-pi./2.0)))./lC))./(lC.*2.0)).*2.0;mlA.*(ddy.*(-1.0./2.0)+(LA.*dq1.^2.*sin(alphaAA-pi./2.0).*cos(q1))./2.0+(LA.*ddq1.*sin(alphaAA-pi./2.0).*sin(q1))./2.0).*(-1.0./2.0)-mlA.*(ddy.*(-1.0./4.0)+(LA.*dq1.^2.*sin(alphaAA-pi./2.0).*cos(q1))./4.0+(LA.*ddq1.*sin(alphaAA-pi./2.0).*sin(q1))./4.0)-(mlB.*(ddy.*(-1.0./2.0)+(LB.*dq2.^2.*sin(alphaAB-pi./2.0).*cos(q2))./2.0+(LB.*ddq2.*sin(alphaAB-pi./2.0).*sin(q2))./2.0))./2.0-mlB.*(ddy.*(-1.0./4.0)+(LB.*dq2.^2.*sin(alphaAB-pi./2.0).*cos(q2))./4.0+(LB.*ddq2.*sin(alphaAB-pi./2.0).*sin(q2))./4.0)-(mlC.*(ddy.*(-1.0./2.0)+(LC.*dq3.^2.*sin(alphaAC-pi./2.0).*cos(q3))./2.0+(LC.*ddq3.*sin(alphaAC-pi./2.0).*sin(q3))./2.0))./2.0-mlC.*(ddy.*(-1.0./4.0)+(LC.*dq3.^2.*sin(alphaAC-pi./2.0).*cos(q3))./4.0+(LC.*ddq3.*sin(alphaAC-pi./2.0).*sin(q3))./4.0)+ddy.*mTCP+(((IlCxz.*1.0./lC.^2.*(dx-LC.*dq3.*sin(q3).*cos(alphaAC-pi./2.0)))./2.0-(IlCxx.*1.0./lC.^2.*(dz+LC.*dq3.*sin(pi./2.0).*cos(q3)))./2.0).*(((dz+LC.*dq3.*sin(pi./2.0).*cos(q3)).*(y+aC.*cos(alphaAC)-eC.*cos(alphaAC)+LC.*cos(alphaAC).*cos(q3)))./lC-((z+LC.*sin(q3)).*(dy+LC.*dq3.*sin(alphaAC-pi./2.0).*sin(q3)))./lC).*2.0)./lC+((((z+LA.*sin(q1)).*(dx-LA.*dq1.*sin(q1).*cos(alphaAA-pi./2.0)))./lA-((dz+LA.*dq1.*sin(pi./2.0).*cos(q1)).*(x+aA.*sin(alphaAA)-eA.*sin(alphaAA)+LA.*cos(q1).*sin(alphaAA)))./lA).*((IlAyz.*1.0./lA.^2.*(dx-LA.*dq1.*sin(q1).*cos(alphaAA-pi./2.0)))./2.0-(IlAxy.*1.0./lA.^2.*(dz+LA.*dq1.*sin(pi./2.0).*cos(q1)))./2.0).*2.0)./lA+((((z+LB.*sin(q2)).*(dx-LB.*dq2.*sin(q2).*cos(alphaAB-pi./2.0)))./lB-((dz+LB.*dq2.*sin(pi./2.0).*cos(q2)).*(x+aB.*sin(alphaAB)-eB.*sin(alphaAB)+LB.*cos(q2).*sin(alphaAB)))./lB).*((IlByz.*1.0./lB.^2.*(dx-LB.*dq2.*sin(q2).*cos(alphaAB-pi./2.0)))./2.0-(IlBxy.*1.0./lB.^2.*(dz+LB.*dq2.*sin(pi./2.0).*cos(q2)))./2.0).*2.0)./lB+((((z+LC.*sin(q3)).*(dx-LC.*dq3.*sin(q3).*cos(alphaAC-pi./2.0)))./lC-((dz+LC.*dq3.*sin(pi./2.0).*cos(q3)).*(x+aC.*sin(alphaAC)-eC.*sin(alphaAC)+LC.*cos(q3).*sin(alphaAC)))./lC).*((IlCyz.*1.0./lC.^2.*(dx-LC.*dq3.*sin(q3).*cos(alphaAC-pi./2.0)))./2.0-(IlCxy.*1.0./lC.^2.*(dz+LC.*dq3.*sin(pi./2.0).*cos(q3)))./2.0).*2.0)./lC+1.0./lA.^2.*(dx-LA.*dq1.*sin(alphaAA).*sin(q1)).*((IlAzz.*(((dx-LA.*dq1.*sin(q1).*cos(alphaAA-pi./2.0)).*(y+aA.*cos(alphaAA)-eA.*cos(alphaAA)+LA.*cos(alphaAA).*cos(q1)))./lA-((dy+LA.*dq1.*sin(alphaAA-pi./2.0).*sin(q1)).*(x+aA.*sin(alphaAA)-eA.*sin(alphaAA)+LA.*cos(q1).*sin(alphaAA)))./lA).*(-1.0./2.0))./lA+(IlAxz.*(((dz+LA.*dq1.*sin(pi./2.0).*cos(q1)).*(y+aA.*cos(alphaAA)-eA.*cos(alphaAA)+LA.*cos(alphaAA).*cos(q1)))./lA-((z+LA.*sin(q1)).*(dy+LA.*dq1.*sin(alphaAA-pi./2.0).*sin(q1)))./lA))./(lA.*2.0)+(IlAyz.*(((z+LA.*sin(q1)).*(dx-LA.*dq1.*sin(q1).*cos(alphaAA-pi./2.0)))./lA-((dz+LA.*dq1.*sin(pi./2.0).*cos(q1)).*(x+aA.*sin(alphaAA)-eA.*sin(alphaAA)+LA.*cos(q1).*sin(alphaAA)))./lA))./(lA.*2.0)).*2.0+1.0./lB.^2.*(dx-LB.*dq2.*sin(alphaAB).*sin(q2)).*((IlBzz.*(((dx-LB.*dq2.*sin(q2).*cos(alphaAB-pi./2.0)).*(y+aB.*cos(alphaAB)-eB.*cos(alphaAB)+LB.*cos(alphaAB).*cos(q2)))./lB-((dy+LB.*dq2.*sin(alphaAB-pi./2.0).*sin(q2)).*(x+aB.*sin(alphaAB)-eB.*sin(alphaAB)+LB.*cos(q2).*sin(alphaAB)))./lB).*(-1.0./2.0))./lB+(IlBxz.*(((dz+LB.*dq2.*sin(pi./2.0).*cos(q2)).*(y+aB.*cos(alphaAB)-eB.*cos(alphaAB)+LB.*cos(alphaAB).*cos(q2)))./lB-((z+LB.*sin(q2)).*(dy+LB.*dq2.*sin(alphaAB-pi./2.0).*sin(q2)))./lB))./(lB.*2.0)+(IlByz.*(((z+LB.*sin(q2)).*(dx-LB.*dq2.*sin(q2).*cos(alphaAB-pi./2.0)))./lB-((dz+LB.*dq2.*sin(pi./2.0).*cos(q2)).*(x+aB.*sin(alphaAB)-eB.*sin(alphaAB)+LB.*cos(q2).*sin(alphaAB)))./lB))./(lB.*2.0)).*2.0+1.0./lC.^2.*(dx-LC.*dq3.*sin(alphaAC).*sin(q3)).*((IlCzz.*(((dx-LC.*dq3.*sin(q3).*cos(alphaAC-pi./2.0)).*(y+aC.*cos(alphaAC)-eC.*cos(alphaAC)+LC.*cos(alphaAC).*cos(q3)))./lC-((dy+LC.*dq3.*sin(alphaAC-pi./2.0).*sin(q3)).*(x+aC.*sin(alphaAC)-eC.*sin(alphaAC)+LC.*cos(q3).*sin(alphaAC)))./lC).*(-1.0./2.0))./lC+(IlCxz.*(((dz+LC.*dq3.*sin(pi./2.0).*cos(q3)).*(y+aC.*cos(alphaAC)-eC.*cos(alphaAC)+LC.*cos(alphaAC).*cos(q3)))./lC-((z+LC.*sin(q3)).*(dy+LC.*dq3.*sin(alphaAC-pi./2.0).*sin(q3)))./lC))./(lC.*2.0)+(IlCyz.*(((z+LC.*sin(q3)).*(dx-LC.*dq3.*sin(q3).*cos(alphaAC-pi./2.0)))./lC-((dz+LC.*dq3.*sin(pi./2.0).*cos(q3)).*(x+aC.*sin(alphaAC)-eC.*sin(alphaAC)+LC.*cos(q3).*sin(alphaAC)))./lC))./(lC.*2.0)).*2.0-(((IlAxz.*1.0./lA.^2.*(x+aA.*sin(alphaAA)-eA.*sin(alphaAA)+LA.*cos(q1).*sin(alphaAA)))./2.0-(IlAxx.*1.0./lA.^2.*(z+LA.*sin(q1)))./2.0).*(((dz+LA.*dq1.*cos(q1)).*(dy+LA.*dq1.*sin(alphaAA-pi./2.0).*sin(q1)))./lA-((dy-LA.*dq1.*cos(alphaAA).*sin(q1)).*(dz+LA.*dq1.*sin(pi./2.0).*cos(q1)))./lA+((z+LA.*sin(q1)).*(ddy+LA.*dq1.^2.*sin(alphaAA-pi./2.0).*cos(q1)+LA.*ddq1.*sin(alphaAA-pi./2.0).*sin(q1)))./lA-((ddz+LA.*ddq1.*sin(pi./2.0).*cos(q1)-LA.*dq1.^2.*sin(pi./2.0).*sin(q1)).*(y+aA.*cos(alphaAA)-eA.*cos(alphaAA)+LA.*cos(alphaAA).*cos(q1)))./lA).*2.0)./lA-(((IlBxz.*1.0./lB.^2.*(x+aB.*sin(alphaAB)-eB.*sin(alphaAB)+LB.*cos(q2).*sin(alphaAB)))./2.0-(IlBxx.*1.0./lB.^2.*(z+LB.*sin(q2)))./2.0).*(((dz+LB.*dq2.*cos(q2)).*(dy+LB.*dq2.*sin(alphaAB-pi./2.0).*sin(q2)))./lB-((dy-LB.*dq2.*cos(alphaAB).*sin(q2)).*(dz+LB.*dq2.*sin(pi./2.0).*cos(q2)))./lB+((z+LB.*sin(q2)).*(ddy+LB.*dq2.^2.*sin(alphaAB-pi./2.0).*cos(q2)+LB.*ddq2.*sin(alphaAB-pi./2.0).*sin(q2)))./lB-((ddz+LB.*ddq2.*sin(pi./2.0).*cos(q2)-LB.*dq2.^2.*sin(pi./2.0).*sin(q2)).*(y+aB.*cos(alphaAB)-eB.*cos(alphaAB)+LB.*cos(alphaAB).*cos(q2)))./lB).*2.0)./lB-(((IlCxz.*1.0./lC.^2.*(x+aC.*sin(alphaAC)-eC.*sin(alphaAC)+LC.*cos(q3).*sin(alphaAC)))./2.0-(IlCxx.*1.0./lC.^2.*(z+LC.*sin(q3)))./2.0).*(((dz+LC.*dq3.*cos(q3)).*(dy+LC.*dq3.*sin(alphaAC-pi./2.0).*sin(q3)))./lC-((dy-LC.*dq3.*cos(alphaAC).*sin(q3)).*(dz+LC.*dq3.*sin(pi./2.0).*cos(q3)))./lC+((z+LC.*sin(q3)).*(ddy+LC.*dq3.^2.*sin(alphaAC-pi./2.0).*cos(q3)+LC.*ddq3.*sin(alphaAC-pi./2.0).*sin(q3)))./lC-((ddz+LC.*ddq3.*sin(pi./2.0).*cos(q3)-LC.*dq3.^2.*sin(pi./2.0).*sin(q3)).*(y+aC.*cos(alphaAC)-eC.*cos(alphaAC)+LC.*cos(alphaAC).*cos(q3)))./lC).*2.0)./lC-1.0./lA.^2.*(dz+LA.*dq1.*cos(q1)).*((IlAxz.*(((dx-LA.*dq1.*sin(q1).*cos(alphaAA-pi./2.0)).*(y+aA.*cos(alphaAA)-eA.*cos(alphaAA)+LA.*cos(alphaAA).*cos(q1)))./lA-((dy+LA.*dq1.*sin(alphaAA-pi./2.0).*sin(q1)).*(x+aA.*sin(alphaAA)-eA.*sin(alphaAA)+LA.*cos(q1).*sin(alphaAA)))./lA).*(-1.0./2.0))./lA+(IlAxx.*(((dz+LA.*dq1.*sin(pi./2.0).*cos(q1)).*(y+aA.*cos(alphaAA)-eA.*cos(alphaAA)+LA.*cos(alphaAA).*cos(q1)))./lA-((z+LA.*sin(q1)).*(dy+LA.*dq1.*sin(alphaAA-pi./2.0).*sin(q1)))./lA))./(lA.*2.0)+(IlAxy.*(((z+LA.*sin(q1)).*(dx-LA.*dq1.*sin(q1).*cos(alphaAA-pi./2.0)))./lA-((dz+LA.*dq1.*sin(pi./2.0).*cos(q1)).*(x+aA.*sin(alphaAA)-eA.*sin(alphaAA)+LA.*cos(q1).*sin(alphaAA)))./lA))./(lA.*2.0)).*2.0-1.0./lB.^2.*(dz+LB.*dq2.*cos(q2)).*((IlBxz.*(((dx-LB.*dq2.*sin(q2).*cos(alphaAB-pi./2.0)).*(y+aB.*cos(alphaAB)-eB.*cos(alphaAB)+LB.*cos(alphaAB).*cos(q2)))./lB-((dy+LB.*dq2.*sin(alphaAB-pi./2.0).*sin(q2)).*(x+aB.*sin(alphaAB)-eB.*sin(alphaAB)+LB.*cos(q2).*sin(alphaAB)))./lB).*(-1.0./2.0))./lB+(IlBxx.*(((dz+LB.*dq2.*sin(pi./2.0).*cos(q2)).*(y+aB.*cos(alphaAB)-eB.*cos(alphaAB)+LB.*cos(alphaAB).*cos(q2)))./lB-((z+LB.*sin(q2)).*(dy+LB.*dq2.*sin(alphaAB-pi./2.0).*sin(q2)))./lB))./(lB.*2.0)+(IlBxy.*(((z+LB.*sin(q2)).*(dx-LB.*dq2.*sin(q2).*cos(alphaAB-pi./2.0)))./lB-((dz+LB.*dq2.*sin(pi./2.0).*cos(q2)).*(x+aB.*sin(alphaAB)-eB.*sin(alphaAB)+LB.*cos(q2).*sin(alphaAB)))./lB))./(lB.*2.0)).*2.0-1.0./lC.^2.*(dz+LC.*dq3.*cos(q3)).*((IlCxz.*(((dx-LC.*dq3.*sin(q3).*cos(alphaAC-pi./2.0)).*(y+aC.*cos(alphaAC)-eC.*cos(alphaAC)+LC.*cos(alphaAC).*cos(q3)))./lC-((dy+LC.*dq3.*sin(alphaAC-pi./2.0).*sin(q3)).*(x+aC.*sin(alphaAC)-eC.*sin(alphaAC)+LC.*cos(q3).*sin(alphaAC)))./lC).*(-1.0./2.0))./lC+(IlCxx.*(((dz+LC.*dq3.*sin(pi./2.0).*cos(q3)).*(y+aC.*cos(alphaAC)-eC.*cos(alphaAC)+LC.*cos(alphaAC).*cos(q3)))./lC-((z+LC.*sin(q3)).*(dy+LC.*dq3.*sin(alphaAC-pi./2.0).*sin(q3)))./lC))./(lC.*2.0)+(IlCxy.*(((z+LC.*sin(q3)).*(dx-LC.*dq3.*sin(q3).*cos(alphaAC-pi./2.0)))./lC-((dz+LC.*dq3.*sin(pi./2.0).*cos(q3)).*(x+aC.*sin(alphaAC)-eC.*sin(alphaAC)+LC.*cos(q3).*sin(alphaAC)))./lC))./(lC.*2.0)).*2.0+1.0./lA.^2.*(dx-LA.*dq1.*sin(q1).*cos(alphaAA-pi./2.0)).*((IlAzz.*(((dx-LA.*dq1.*sin(q1).*cos(alphaAA-pi./2.0)).*(y+aA.*cos(alphaAA)-eA.*cos(alphaAA)+LA.*cos(alphaAA).*cos(q1)))./lA-((dy+LA.*dq1.*sin(alphaAA-pi./2.0).*sin(q1)).*(x+aA.*sin(alphaAA)-eA.*sin(alphaAA)+LA.*cos(q1).*sin(alphaAA)))./lA).*(-1.0./2.0))./lA+(IlAxz.*(((dz+LA.*dq1.*sin(pi./2.0).*cos(q1)).*(y+aA.*cos(alphaAA)-eA.*cos(alphaAA)+LA.*cos(alphaAA).*cos(q1)))./lA-((z+LA.*sin(q1)).*(dy+LA.*dq1.*sin(alphaAA-pi./2.0).*sin(q1)))./lA))./(lA.*2.0)+(IlAyz.*(((z+LA.*sin(q1)).*(dx-LA.*dq1.*sin(q1).*cos(alphaAA-pi./2.0)))./lA-((dz+LA.*dq1.*sin(pi./2.0).*cos(q1)).*(x+aA.*sin(alphaAA)-eA.*sin(alphaAA)+LA.*cos(q1).*sin(alphaAA)))./lA))./(lA.*2.0)).*2.0+1.0./lB.^2.*(dx-LB.*dq2.*sin(q2).*cos(alphaAB-pi./2.0)).*((IlBzz.*(((dx-LB.*dq2.*sin(q2).*cos(alphaAB-pi./2.0)).*(y+aB.*cos(alphaAB)-eB.*cos(alphaAB)+LB.*cos(alphaAB).*cos(q2)))./lB-((dy+LB.*dq2.*sin(alphaAB-pi./2.0).*sin(q2)).*(x+aB.*sin(alphaAB)-eB.*sin(alphaAB)+LB.*cos(q2).*sin(alphaAB)))./lB).*(-1.0./2.0))./lB+(IlBxz.*(((dz+LB.*dq2.*sin(pi./2.0).*cos(q2)).*(y+aB.*cos(alphaAB)-eB.*cos(alphaAB)+LB.*cos(alphaAB).*cos(q2)))./lB-((z+LB.*sin(q2)).*(dy+LB.*dq2.*sin(alphaAB-pi./2.0).*sin(q2)))./lB))./(lB.*2.0)+(IlByz.*(((z+LB.*sin(q2)).*(dx-LB.*dq2.*sin(q2).*cos(alphaAB-pi./2.0)))./lB-((dz+LB.*dq2.*sin(pi./2.0).*cos(q2)).*(x+aB.*sin(alphaAB)-eB.*sin(alphaAB)+LB.*cos(q2).*sin(alphaAB)))./lB))./(lB.*2.0)).*2.0+1.0./lC.^2.*(dx-LC.*dq3.*sin(q3).*cos(alphaAC-pi./2.0)).*((IlCzz.*(((dx-LC.*dq3.*sin(q3).*cos(alphaAC-pi./2.0)).*(y+aC.*cos(alphaAC)-eC.*cos(alphaAC)+LC.*cos(alphaAC).*cos(q3)))./lC-((dy+LC.*dq3.*sin(alphaAC-pi./2.0).*sin(q3)).*(x+aC.*sin(alphaAC)-eC.*sin(alphaAC)+LC.*cos(q3).*sin(alphaAC)))./lC).*(-1.0./2.0))./lC+(IlCxz.*(((dz+LC.*dq3.*sin(pi./2.0).*cos(q3)).*(y+aC.*cos(alphaAC)-eC.*cos(alphaAC)+LC.*cos(alphaAC).*cos(q3)))./lC-((z+LC.*sin(q3)).*(dy+LC.*dq3.*sin(alphaAC-pi./2.0).*sin(q3)))./lC))./(lC.*2.0)+(IlCyz.*(((z+LC.*sin(q3)).*(dx-LC.*dq3.*sin(q3).*cos(alphaAC-pi./2.0)))./lC-((dz+LC.*dq3.*sin(pi./2.0).*cos(q3)).*(x+aC.*sin(alphaAC)-eC.*sin(alphaAC)+LC.*cos(q3).*sin(alphaAC)))./lC))./(lC.*2.0)).*2.0-(((IlAzz.*1.0./lA.^2.*(dx-LA.*dq1.*sin(alphaAA).*sin(q1)))./2.0-(IlAxz.*1.0./lA.^2.*(dz+LA.*dq1.*cos(q1)))./2.0).*(((dx-LA.*dq1.*sin(q1).*cos(alphaAA-pi./2.0)).*(y+aA.*cos(alphaAA)-eA.*cos(alphaAA)+LA.*cos(alphaAA).*cos(q1)))./lA-((dy+LA.*dq1.*sin(alphaAA-pi./2.0).*sin(q1)).*(x+aA.*sin(alphaAA)-eA.*sin(alphaAA)+LA.*cos(q1).*sin(alphaAA)))./lA).*2.0)./lA-(((IlBzz.*1.0./lB.^2.*(dx-LB.*dq2.*sin(alphaAB).*sin(q2)))./2.0-(IlBxz.*1.0./lB.^2.*(dz+LB.*dq2.*cos(q2)))./2.0).*(((dx-LB.*dq2.*sin(q2).*cos(alphaAB-pi./2.0)).*(y+aB.*cos(alphaAB)-eB.*cos(alphaAB)+LB.*cos(alphaAB).*cos(q2)))./lB-((dy+LB.*dq2.*sin(alphaAB-pi./2.0).*sin(q2)).*(x+aB.*sin(alphaAB)-eB.*sin(alphaAB)+LB.*cos(q2).*sin(alphaAB)))./lB).*2.0)./lB-(((IlCzz.*1.0./lC.^2.*(dx-LC.*dq3.*sin(alphaAC).*sin(q3)))./2.0-(IlCxz.*1.0./lC.^2.*(dz+LC.*dq3.*cos(q3)))./2.0).*(((dx-LC.*dq3.*sin(q3).*cos(alphaAC-pi./2.0)).*(y+aC.*cos(alphaAC)-eC.*cos(alphaAC)+LC.*cos(alphaAC).*cos(q3)))./lC-((dy+LC.*dq3.*sin(alphaAC-pi./2.0).*sin(q3)).*(x+aC.*sin(alphaAC)-eC.*sin(alphaAC)+LC.*cos(q3).*sin(alphaAC)))./lC).*2.0)./lC-1.0./lA.^2.*(dz+LA.*dq1.*sin(pi./2.0).*cos(q1)).*((IlAxz.*(((dx-LA.*dq1.*sin(q1).*cos(alphaAA-pi./2.0)).*(y+aA.*cos(alphaAA)-eA.*cos(alphaAA)+LA.*cos(alphaAA).*cos(q1)))./lA-((dy+LA.*dq1.*sin(alphaAA-pi./2.0).*sin(q1)).*(x+aA.*sin(alphaAA)-eA.*sin(alphaAA)+LA.*cos(q1).*sin(alphaAA)))./lA).*(-1.0./2.0))./lA+(IlAxx.*(((dz+LA.*dq1.*sin(pi./2.0).*cos(q1)).*(y+aA.*cos(alphaAA)-eA.*cos(alphaAA)+LA.*cos(alphaAA).*cos(q1)))./lA-((z+LA.*sin(q1)).*(dy+LA.*dq1.*sin(alphaAA-pi./2.0).*sin(q1)))./lA))./(lA.*2.0)+(IlAxy.*(((z+LA.*sin(q1)).*(dx-LA.*dq1.*sin(q1).*cos(alphaAA-pi./2.0)))./lA-((dz+LA.*dq1.*sin(pi./2.0).*cos(q1)).*(x+aA.*sin(alphaAA)-eA.*sin(alphaAA)+LA.*cos(q1).*sin(alphaAA)))./lA))./(lA.*2.0)).*2.0-1.0./lB.^2.*(dz+LB.*dq2.*sin(pi./2.0).*cos(q2)).*((IlBxz.*(((dx-LB.*dq2.*sin(q2).*cos(alphaAB-pi./2.0)).*(y+aB.*cos(alphaAB)-eB.*cos(alphaAB)+LB.*cos(alphaAB).*cos(q2)))./lB-((dy+LB.*dq2.*sin(alphaAB-pi./2.0).*sin(q2)).*(x+aB.*sin(alphaAB)-eB.*sin(alphaAB)+LB.*cos(q2).*sin(alphaAB)))./lB).*(-1.0./2.0))./lB+(IlBxx.*(((dz+LB.*dq2.*sin(pi./2.0).*cos(q2)).*(y+aB.*cos(alphaAB)-eB.*cos(alphaAB)+LB.*cos(alphaAB).*cos(q2)))./lB-((z+LB.*sin(q2)).*(dy+LB.*dq2.*sin(alphaAB-pi./2.0).*sin(q2)))./lB))./(lB.*2.0)+(IlBxy.*(((z+LB.*sin(q2)).*(dx-LB.*dq2.*sin(q2).*cos(alphaAB-pi./2.0)))./lB-((dz+LB.*dq2.*sin(pi./2.0).*cos(q2)).*(x+aB.*sin(alphaAB)-eB.*sin(alphaAB)+LB.*cos(q2).*sin(alphaAB)))./lB))./(lB.*2.0)).*2.0-1.0./lC.^2.*(dz+LC.*dq3.*sin(pi./2.0).*cos(q3)).*((IlCxz.*(((dx-LC.*dq3.*sin(q3).*cos(alphaAC-pi./2.0)).*(y+aC.*cos(alphaAC)-eC.*cos(alphaAC)+LC.*cos(alphaAC).*cos(q3)))./lC-((dy+LC.*dq3.*sin(alphaAC-pi./2.0).*sin(q3)).*(x+aC.*sin(alphaAC)-eC.*sin(alphaAC)+LC.*cos(q3).*sin(alphaAC)))./lC).*(-1.0./2.0))./lC+(IlCxx.*(((dz+LC.*dq3.*sin(pi./2.0).*cos(q3)).*(y+aC.*cos(alphaAC)-eC.*cos(alphaAC)+LC.*cos(alphaAC).*cos(q3)))./lC-((z+LC.*sin(q3)).*(dy+LC.*dq3.*sin(alphaAC-pi./2.0).*sin(q3)))./lC))./(lC.*2.0)+(IlCxy.*(((z+LC.*sin(q3)).*(dx-LC.*dq3.*sin(q3).*cos(alphaAC-pi./2.0)))./lC-((dz+LC.*dq3.*sin(pi./2.0).*cos(q3)).*(x+aC.*sin(alphaAC)-eC.*sin(alphaAC)+LC.*cos(q3).*sin(alphaAC)))./lC))./(lC.*2.0)).*2.0+(((IlAzz.*1.0./lA.^2.*(x+aA.*sin(alphaAA)-eA.*sin(alphaAA)+LA.*cos(q1).*sin(alphaAA)))./2.0-(IlAxz.*1.0./lA.^2.*(z+LA.*sin(q1)))./2.0).*(-((dy-LA.*dq1.*cos(alphaAA).*sin(q1)).*(dx-LA.*dq1.*sin(q1).*cos(alphaAA-pi./2.0)))./lA+((dx-LA.*dq1.*sin(alphaAA).*sin(q1)).*(dy+LA.*dq1.*sin(alphaAA-pi./2.0).*sin(q1)))./lA+((ddy+LA.*dq1.^2.*sin(alphaAA-pi./2.0).*cos(q1)+LA.*ddq1.*sin(alphaAA-pi./2.0).*sin(q1)).*(x+aA.*sin(alphaAA)-eA.*sin(alphaAA)+LA.*cos(q1).*sin(alphaAA)))./lA+((-ddx+LA.*dq1.^2.*cos(q1).*cos(alphaAA-pi./2.0)+LA.*ddq1.*sin(q1).*cos(alphaAA-pi./2.0)).*(y+aA.*cos(alphaAA)-eA.*cos(alphaAA)+LA.*cos(alphaAA).*cos(q1)))./lA).*2.0)./lA+(((IlBzz.*1.0./lB.^2.*(x+aB.*sin(alphaAB)-eB.*sin(alphaAB)+LB.*cos(q2).*sin(alphaAB)))./2.0-(IlBxz.*1.0./lB.^2.*(z+LB.*sin(q2)))./2.0).*(-((dy-LB.*dq2.*cos(alphaAB).*sin(q2)).*(dx-LB.*dq2.*sin(q2).*cos(alphaAB-pi./2.0)))./lB+((dx-LB.*dq2.*sin(alphaAB).*sin(q2)).*(dy+LB.*dq2.*sin(alphaAB-pi./2.0).*sin(q2)))./lB+((ddy+LB.*dq2.^2.*sin(alphaAB-pi./2.0).*cos(q2)+LB.*ddq2.*sin(alphaAB-pi./2.0).*sin(q2)).*(x+aB.*sin(alphaAB)-eB.*sin(alphaAB)+LB.*cos(q2).*sin(alphaAB)))./lB+((-ddx+LB.*dq2.^2.*cos(q2).*cos(alphaAB-pi./2.0)+LB.*ddq2.*sin(q2).*cos(alphaAB-pi./2.0)).*(y+aB.*cos(alphaAB)-eB.*cos(alphaAB)+LB.*cos(alphaAB).*cos(q2)))./lB).*2.0)./lB+(((IlCzz.*1.0./lC.^2.*(x+aC.*sin(alphaAC)-eC.*sin(alphaAC)+LC.*cos(q3).*sin(alphaAC)))./2.0-(IlCxz.*1.0./lC.^2.*(z+LC.*sin(q3)))./2.0).*(-((dy-LC.*dq3.*cos(alphaAC).*sin(q3)).*(dx-LC.*dq3.*sin(q3).*cos(alphaAC-pi./2.0)))./lC+((dx-LC.*dq3.*sin(alphaAC).*sin(q3)).*(dy+LC.*dq3.*sin(alphaAC-pi./2.0).*sin(q3)))./lC+((ddy+LC.*dq3.^2.*sin(alphaAC-pi./2.0).*cos(q3)+LC.*ddq3.*sin(alphaAC-pi./2.0).*sin(q3)).*(x+aC.*sin(alphaAC)-eC.*sin(alphaAC)+LC.*cos(q3).*sin(alphaAC)))./lC+((-ddx+LC.*dq3.^2.*cos(q3).*cos(alphaAC-pi./2.0)+LC.*ddq3.*sin(q3).*cos(alphaAC-pi./2.0)).*(y+aC.*cos(alphaAC)-eC.*cos(alphaAC)+LC.*cos(alphaAC).*cos(q3)))./lC).*2.0)./lC+(((IlAxz.*1.0./lA.^2.*(dx-LA.*dq1.*sin(alphaAA).*sin(q1)))./2.0-(IlAxx.*1.0./lA.^2.*(dz+LA.*dq1.*cos(q1)))./2.0).*(((dz+LA.*dq1.*sin(pi./2.0).*cos(q1)).*(y+aA.*cos(alphaAA)-eA.*cos(alphaAA)+LA.*cos(alphaAA).*cos(q1)))./lA-((z+LA.*sin(q1)).*(dy+LA.*dq1.*sin(alphaAA-pi./2.0).*sin(q1)))./lA).*2.0)./lA+(((IlBxz.*1.0./lB.^2.*(dx-LB.*dq2.*sin(alphaAB).*sin(q2)))./2.0-(IlBxx.*1.0./lB.^2.*(dz+LB.*dq2.*cos(q2)))./2.0).*(((dz+LB.*dq2.*sin(pi./2.0).*cos(q2)).*(y+aB.*cos(alphaAB)-eB.*cos(alphaAB)+LB.*cos(alphaAB).*cos(q2)))./lB-((z+LB.*sin(q2)).*(dy+LB.*dq2.*sin(alphaAB-pi./2.0).*sin(q2)))./lB).*2.0)./lB+(((IlCxz.*1.0./lC.^2.*(dx-LC.*dq3.*sin(alphaAC).*sin(q3)))./2.0-(IlCxx.*1.0./lC.^2.*(dz+LC.*dq3.*cos(q3)))./2.0).*(((dz+LC.*dq3.*sin(pi./2.0).*cos(q3)).*(y+aC.*cos(alphaAC)-eC.*cos(alphaAC)+LC.*cos(alphaAC).*cos(q3)))./lC-((z+LC.*sin(q3)).*(dy+LC.*dq3.*sin(alphaAC-pi./2.0).*sin(q3)))./lC).*2.0)./lC-(((IlAyz.*1.0./lA.^2.*(x+aA.*sin(alphaAA)-eA.*sin(alphaAA)+LA.*cos(q1).*sin(alphaAA)))./2.0-(IlAxy.*1.0./lA.^2.*(z+LA.*sin(q1)))./2.0).*(((ddz+LA.*ddq1.*sin(pi./2.0).*cos(q1)-LA.*dq1.^2.*sin(pi./2.0).*sin(q1)).*(x+aA.*sin(alphaAA)-eA.*sin(alphaAA)+LA.*cos(q1).*sin(alphaAA)))./lA-((dz+LA.*dq1.*cos(q1)).*(dx-LA.*dq1.*sin(q1).*cos(alphaAA-pi./2.0)))./lA+((dx-LA.*dq1.*sin(alphaAA).*sin(q1)).*(dz+LA.*dq1.*sin(pi./2.0).*cos(q1)))./lA+((z+LA.*sin(q1)).*(-ddx+LA.*dq1.^2.*cos(q1).*cos(alphaAA-pi./2.0)+LA.*ddq1.*sin(q1).*cos(alphaAA-pi./2.0)))./lA).*2.0)./lA-(((IlByz.*1.0./lB.^2.*(x+aB.*sin(alphaAB)-eB.*sin(alphaAB)+LB.*cos(q2).*sin(alphaAB)))./2.0-(IlBxy.*1.0./lB.^2.*(z+LB.*sin(q2)))./2.0).*(((ddz+LB.*ddq2.*sin(pi./2.0).*cos(q2)-LB.*dq2.^2.*sin(pi./2.0).*sin(q2)).*(x+aB.*sin(alphaAB)-eB.*sin(alphaAB)+LB.*cos(q2).*sin(alphaAB)))./lB-((dz+LB.*dq2.*cos(q2)).*(dx-LB.*dq2.*sin(q2).*cos(alphaAB-pi./2.0)))./lB+((dx-LB.*dq2.*sin(alphaAB).*sin(q2)).*(dz+LB.*dq2.*sin(pi./2.0).*cos(q2)))./lB+((z+LB.*sin(q2)).*(-ddx+LB.*dq2.^2.*cos(q2).*cos(alphaAB-pi./2.0)+LB.*ddq2.*sin(q2).*cos(alphaAB-pi./2.0)))./lB).*2.0)./lB-(((IlCyz.*1.0./lC.^2.*(x+aC.*sin(alphaAC)-eC.*sin(alphaAC)+LC.*cos(q3).*sin(alphaAC)))./2.0-(IlCxy.*1.0./lC.^2.*(z+LC.*sin(q3)))./2.0).*(((ddz+LC.*ddq3.*sin(pi./2.0).*cos(q3)-LC.*dq3.^2.*sin(pi./2.0).*sin(q3)).*(x+aC.*sin(alphaAC)-eC.*sin(alphaAC)+LC.*cos(q3).*sin(alphaAC)))./lC-((dz+LC.*dq3.*cos(q3)).*(dx-LC.*dq3.*sin(q3).*cos(alphaAC-pi./2.0)))./lC+((dx-LC.*dq3.*sin(alphaAC).*sin(q3)).*(dz+LC.*dq3.*sin(pi./2.0).*cos(q3)))./lC+((z+LC.*sin(q3)).*(-ddx+LC.*dq3.^2.*cos(q3).*cos(alphaAC-pi./2.0)+LC.*ddq3.*sin(q3).*cos(alphaAC-pi./2.0)))./lC).*2.0)./lC-((((dx-LA.*dq1.*sin(q1).*cos(alphaAA-pi./2.0)).*(y+aA.*cos(alphaAA)-eA.*cos(alphaAA)+LA.*cos(alphaAA).*cos(q1)))./lA-((dy+LA.*dq1.*sin(alphaAA-pi./2.0).*sin(q1)).*(x+aA.*sin(alphaAA)-eA.*sin(alphaAA)+LA.*cos(q1).*sin(alphaAA)))./lA).*((IlAzz.*1.0./lA.^2.*(dx-LA.*dq1.*sin(q1).*cos(alphaAA-pi./2.0)))./2.0-(IlAxz.*1.0./lA.^2.*(dz+LA.*dq1.*sin(pi./2.0).*cos(q1)))./2.0).*2.0)./lA-((((dx-LB.*dq2.*sin(q2).*cos(alphaAB-pi./2.0)).*(y+aB.*cos(alphaAB)-eB.*cos(alphaAB)+LB.*cos(alphaAB).*cos(q2)))./lB-((dy+LB.*dq2.*sin(alphaAB-pi./2.0).*sin(q2)).*(x+aB.*sin(alphaAB)-eB.*sin(alphaAB)+LB.*cos(q2).*sin(alphaAB)))./lB).*((IlBzz.*1.0./lB.^2.*(dx-LB.*dq2.*sin(q2).*cos(alphaAB-pi./2.0)))./2.0-(IlBxz.*1.0./lB.^2.*(dz+LB.*dq2.*sin(pi./2.0).*cos(q2)))./2.0).*2.0)./lB-((((dx-LC.*dq3.*sin(q3).*cos(alphaAC-pi./2.0)).*(y+aC.*cos(alphaAC)-eC.*cos(alphaAC)+LC.*cos(alphaAC).*cos(q3)))./lC-((dy+LC.*dq3.*sin(alphaAC-pi./2.0).*sin(q3)).*(x+aC.*sin(alphaAC)-eC.*sin(alphaAC)+LC.*cos(q3).*sin(alphaAC)))./lC).*((IlCzz.*1.0./lC.^2.*(dx-LC.*dq3.*sin(q3).*cos(alphaAC-pi./2.0)))./2.0-(IlCxz.*1.0./lC.^2.*(dz+LC.*dq3.*sin(pi./2.0).*cos(q3)))./2.0).*2.0)./lC+((((z+LA.*sin(q1)).*(dx-LA.*dq1.*sin(q1).*cos(alphaAA-pi./2.0)))./lA-((dz+LA.*dq1.*sin(pi./2.0).*cos(q1)).*(x+aA.*sin(alphaAA)-eA.*sin(alphaAA)+LA.*cos(q1).*sin(alphaAA)))./lA).*((IlAyz.*1.0./lA.^2.*(dx-LA.*dq1.*sin(alphaAA).*sin(q1)))./2.0-(IlAxy.*1.0./lA.^2.*(dz+LA.*dq1.*cos(q1)))./2.0).*2.0)./lA+((((z+LB.*sin(q2)).*(dx-LB.*dq2.*sin(q2).*cos(alphaAB-pi./2.0)))./lB-((dz+LB.*dq2.*sin(pi./2.0).*cos(q2)).*(x+aB.*sin(alphaAB)-eB.*sin(alphaAB)+LB.*cos(q2).*sin(alphaAB)))./lB).*((IlByz.*1.0./lB.^2.*(dx-LB.*dq2.*sin(alphaAB).*sin(q2)))./2.0-(IlBxy.*1.0./lB.^2.*(dz+LB.*dq2.*cos(q2)))./2.0).*2.0)./lB+((((z+LC.*sin(q3)).*(dx-LC.*dq3.*sin(q3).*cos(alphaAC-pi./2.0)))./lC-((dz+LC.*dq3.*sin(pi./2.0).*cos(q3)).*(x+aC.*sin(alphaAC)-eC.*sin(alphaAC)+LC.*cos(q3).*sin(alphaAC)))./lC).*((IlCyz.*1.0./lC.^2.*(dx-LC.*dq3.*sin(alphaAC).*sin(q3)))./2.0-(IlCxy.*1.0./lC.^2.*(dz+LC.*dq3.*cos(q3)))./2.0).*2.0)./lC-1.0./lA.^2.*((IlAxz.*(((dz+LA.*dq1.*cos(q1)).*(dy+LA.*dq1.*sin(alphaAA-pi./2.0).*sin(q1)))./lA-((dy-LA.*dq1.*cos(alphaAA).*sin(q1)).*(dz+LA.*dq1.*sin(pi./2.0).*cos(q1)))./lA+((z+LA.*sin(q1)).*(ddy+LA.*dq1.^2.*sin(alphaAA-pi./2.0).*cos(q1)+LA.*ddq1.*sin(alphaAA-pi./2.0).*sin(q1)))./lA-((ddz+LA.*ddq1.*sin(pi./2.0).*cos(q1)-LA.*dq1.^2.*sin(pi./2.0).*sin(q1)).*(y+aA.*cos(alphaAA)-eA.*cos(alphaAA)+LA.*cos(alphaAA).*cos(q1)))./lA))./(lA.*2.0)-(IlAzz.*(-((dy-LA.*dq1.*cos(alphaAA).*sin(q1)).*(dx-LA.*dq1.*sin(q1).*cos(alphaAA-pi./2.0)))./lA+((dx-LA.*dq1.*sin(alphaAA).*sin(q1)).*(dy+LA.*dq1.*sin(alphaAA-pi./2.0).*sin(q1)))./lA+((ddy+LA.*dq1.^2.*sin(alphaAA-pi./2.0).*cos(q1)+LA.*ddq1.*sin(alphaAA-pi./2.0).*sin(q1)).*(x+aA.*sin(alphaAA)-eA.*sin(alphaAA)+LA.*cos(q1).*sin(alphaAA)))./lA+((-ddx+LA.*dq1.^2.*cos(q1).*cos(alphaAA-pi./2.0)+LA.*ddq1.*sin(q1).*cos(alphaAA-pi./2.0)).*(y+aA.*cos(alphaAA)-eA.*cos(alphaAA)+LA.*cos(alphaAA).*cos(q1)))./lA))./(lA.*2.0)+(IlAyz.*(((ddz+LA.*ddq1.*sin(pi./2.0).*cos(q1)-LA.*dq1.^2.*sin(pi./2.0).*sin(q1)).*(x+aA.*sin(alphaAA)-eA.*sin(alphaAA)+LA.*cos(q1).*sin(alphaAA)))./lA-((dz+LA.*dq1.*cos(q1)).*(dx-LA.*dq1.*sin(q1).*cos(alphaAA-pi./2.0)))./lA+((dx-LA.*dq1.*sin(alphaAA).*sin(q1)).*(dz+LA.*dq1.*sin(pi./2.0).*cos(q1)))./lA+((z+LA.*sin(q1)).*(-ddx+LA.*dq1.^2.*cos(q1).*cos(alphaAA-pi./2.0)+LA.*ddq1.*sin(q1).*cos(alphaAA-pi./2.0)))./lA))./(lA.*2.0)).*(x+aA.*sin(alphaAA)-eA.*sin(alphaAA)+LA.*cos(q1).*sin(alphaAA)).*2.0-1.0./lB.^2.*((IlBxz.*(((dz+LB.*dq2.*cos(q2)).*(dy+LB.*dq2.*sin(alphaAB-pi./2.0).*sin(q2)))./lB-((dy-LB.*dq2.*cos(alphaAB).*sin(q2)).*(dz+LB.*dq2.*sin(pi./2.0).*cos(q2)))./lB+((z+LB.*sin(q2)).*(ddy+LB.*dq2.^2.*sin(alphaAB-pi./2.0).*cos(q2)+LB.*ddq2.*sin(alphaAB-pi./2.0).*sin(q2)))./lB-((ddz+LB.*ddq2.*sin(pi./2.0).*cos(q2)-LB.*dq2.^2.*sin(pi./2.0).*sin(q2)).*(y+aB.*cos(alphaAB)-eB.*cos(alphaAB)+LB.*cos(alphaAB).*cos(q2)))./lB))./(lB.*2.0)-(IlBzz.*(-((dy-LB.*dq2.*cos(alphaAB).*sin(q2)).*(dx-LB.*dq2.*sin(q2).*cos(alphaAB-pi./2.0)))./lB+((dx-LB.*dq2.*sin(alphaAB).*sin(q2)).*(dy+LB.*dq2.*sin(alphaAB-pi./2.0).*sin(q2)))./lB+((ddy+LB.*dq2.^2.*sin(alphaAB-pi./2.0).*cos(q2)+LB.*ddq2.*sin(alphaAB-pi./2.0).*sin(q2)).*(x+aB.*sin(alphaAB)-eB.*sin(alphaAB)+LB.*cos(q2).*sin(alphaAB)))./lB+((-ddx+LB.*dq2.^2.*cos(q2).*cos(alphaAB-pi./2.0)+LB.*ddq2.*sin(q2).*cos(alphaAB-pi./2.0)).*(y+aB.*cos(alphaAB)-eB.*cos(alphaAB)+LB.*cos(alphaAB).*cos(q2)))./lB))./(lB.*2.0)+(IlByz.*(((ddz+LB.*ddq2.*sin(pi./2.0).*cos(q2)-LB.*dq2.^2.*sin(pi./2.0).*sin(q2)).*(x+aB.*sin(alphaAB)-eB.*sin(alphaAB)+LB.*cos(q2).*sin(alphaAB)))./lB-((dz+LB.*dq2.*cos(q2)).*(dx-LB.*dq2.*sin(q2).*cos(alphaAB-pi./2.0)))./lB+((dx-LB.*dq2.*sin(alphaAB).*sin(q2)).*(dz+LB.*dq2.*sin(pi./2.0).*cos(q2)))./lB+((z+LB.*sin(q2)).*(-ddx+LB.*dq2.^2.*cos(q2).*cos(alphaAB-pi./2.0)+LB.*ddq2.*sin(q2).*cos(alphaAB-pi./2.0)))./lB))./(lB.*2.0)).*(x+aB.*sin(alphaAB)-eB.*sin(alphaAB)+LB.*cos(q2).*sin(alphaAB)).*2.0-1.0./lC.^2.*((IlCxz.*(((dz+LC.*dq3.*cos(q3)).*(dy+LC.*dq3.*sin(alphaAC-pi./2.0).*sin(q3)))./lC-((dy-LC.*dq3.*cos(alphaAC).*sin(q3)).*(dz+LC.*dq3.*sin(pi./2.0).*cos(q3)))./lC+((z+LC.*sin(q3)).*(ddy+LC.*dq3.^2.*sin(alphaAC-pi./2.0).*cos(q3)+LC.*ddq3.*sin(alphaAC-pi./2.0).*sin(q3)))./lC-((ddz+LC.*ddq3.*sin(pi./2.0).*cos(q3)-LC.*dq3.^2.*sin(pi./2.0).*sin(q3)).*(y+aC.*cos(alphaAC)-eC.*cos(alphaAC)+LC.*cos(alphaAC).*cos(q3)))./lC))./(lC.*2.0)-(IlCzz.*(-((dy-LC.*dq3.*cos(alphaAC).*sin(q3)).*(dx-LC.*dq3.*sin(q3).*cos(alphaAC-pi./2.0)))./lC+((dx-LC.*dq3.*sin(alphaAC).*sin(q3)).*(dy+LC.*dq3.*sin(alphaAC-pi./2.0).*sin(q3)))./lC+((ddy+LC.*dq3.^2.*sin(alphaAC-pi./2.0).*cos(q3)+LC.*ddq3.*sin(alphaAC-pi./2.0).*sin(q3)).*(x+aC.*sin(alphaAC)-eC.*sin(alphaAC)+LC.*cos(q3).*sin(alphaAC)))./lC+((-ddx+LC.*dq3.^2.*cos(q3).*cos(alphaAC-pi./2.0)+LC.*ddq3.*sin(q3).*cos(alphaAC-pi./2.0)).*(y+aC.*cos(alphaAC)-eC.*cos(alphaAC)+LC.*cos(alphaAC).*cos(q3)))./lC))./(lC.*2.0)+(IlCyz.*(((ddz+LC.*ddq3.*sin(pi./2.0).*cos(q3)-LC.*dq3.^2.*sin(pi./2.0).*sin(q3)).*(x+aC.*sin(alphaAC)-eC.*sin(alphaAC)+LC.*cos(q3).*sin(alphaAC)))./lC-((dz+LC.*dq3.*cos(q3)).*(dx-LC.*dq3.*sin(q3).*cos(alphaAC-pi./2.0)))./lC+((dx-LC.*dq3.*sin(alphaAC).*sin(q3)).*(dz+LC.*dq3.*sin(pi./2.0).*cos(q3)))./lC+((z+LC.*sin(q3)).*(-ddx+LC.*dq3.^2.*cos(q3).*cos(alphaAC-pi./2.0)+LC.*ddq3.*sin(q3).*cos(alphaAC-pi./2.0)))./lC))./(lC.*2.0)).*(x+aC.*sin(alphaAC)-eC.*sin(alphaAC)+LC.*cos(q3).*sin(alphaAC)).*2.0+1.0./lA.^2.*(z+LA.*sin(q1)).*((IlAxx.*(((dz+LA.*dq1.*cos(q1)).*(dy+LA.*dq1.*sin(alphaAA-pi./2.0).*sin(q1)))./lA-((dy-LA.*dq1.*cos(alphaAA).*sin(q1)).*(dz+LA.*dq1.*sin(pi./2.0).*cos(q1)))./lA+((z+LA.*sin(q1)).*(ddy+LA.*dq1.^2.*sin(alphaAA-pi./2.0).*cos(q1)+LA.*ddq1.*sin(alphaAA-pi./2.0).*sin(q1)))./lA-((ddz+LA.*ddq1.*sin(pi./2.0).*cos(q1)-LA.*dq1.^2.*sin(pi./2.0).*sin(q1)).*(y+aA.*cos(alphaAA)-eA.*cos(alphaAA)+LA.*cos(alphaAA).*cos(q1)))./lA))./(lA.*2.0)-(IlAxz.*(-((dy-LA.*dq1.*cos(alphaAA).*sin(q1)).*(dx-LA.*dq1.*sin(q1).*cos(alphaAA-pi./2.0)))./lA+((dx-LA.*dq1.*sin(alphaAA).*sin(q1)).*(dy+LA.*dq1.*sin(alphaAA-pi./2.0).*sin(q1)))./lA+((ddy+LA.*dq1.^2.*sin(alphaAA-pi./2.0).*cos(q1)+LA.*ddq1.*sin(alphaAA-pi./2.0).*sin(q1)).*(x+aA.*sin(alphaAA)-eA.*sin(alphaAA)+LA.*cos(q1).*sin(alphaAA)))./lA+((-ddx+LA.*dq1.^2.*cos(q1).*cos(alphaAA-pi./2.0)+LA.*ddq1.*sin(q1).*cos(alphaAA-pi./2.0)).*(y+aA.*cos(alphaAA)-eA.*cos(alphaAA)+LA.*cos(alphaAA).*cos(q1)))./lA))./(lA.*2.0)+(IlAxy.*(((ddz+LA.*ddq1.*sin(pi./2.0).*cos(q1)-LA.*dq1.^2.*sin(pi./2.0).*sin(q1)).*(x+aA.*sin(alphaAA)-eA.*sin(alphaAA)+LA.*cos(q1).*sin(alphaAA)))./lA-((dz+LA.*dq1.*cos(q1)).*(dx-LA.*dq1.*sin(q1).*cos(alphaAA-pi./2.0)))./lA+((dx-LA.*dq1.*sin(alphaAA).*sin(q1)).*(dz+LA.*dq1.*sin(pi./2.0).*cos(q1)))./lA+((z+LA.*sin(q1)).*(-ddx+LA.*dq1.^2.*cos(q1).*cos(alphaAA-pi./2.0)+LA.*ddq1.*sin(q1).*cos(alphaAA-pi./2.0)))./lA))./(lA.*2.0)).*2.0+1.0./lB.^2.*(z+LB.*sin(q2)).*((IlBxx.*(((dz+LB.*dq2.*cos(q2)).*(dy+LB.*dq2.*sin(alphaAB-pi./2.0).*sin(q2)))./lB-((dy-LB.*dq2.*cos(alphaAB).*sin(q2)).*(dz+LB.*dq2.*sin(pi./2.0).*cos(q2)))./lB+((z+LB.*sin(q2)).*(ddy+LB.*dq2.^2.*sin(alphaAB-pi./2.0).*cos(q2)+LB.*ddq2.*sin(alphaAB-pi./2.0).*sin(q2)))./lB-((ddz+LB.*ddq2.*sin(pi./2.0).*cos(q2)-LB.*dq2.^2.*sin(pi./2.0).*sin(q2)).*(y+aB.*cos(alphaAB)-eB.*cos(alphaAB)+LB.*cos(alphaAB).*cos(q2)))./lB))./(lB.*2.0)-(IlBxz.*(-((dy-LB.*dq2.*cos(alphaAB).*sin(q2)).*(dx-LB.*dq2.*sin(q2).*cos(alphaAB-pi./2.0)))./lB+((dx-LB.*dq2.*sin(alphaAB).*sin(q2)).*(dy+LB.*dq2.*sin(alphaAB-pi./2.0).*sin(q2)))./lB+((ddy+LB.*dq2.^2.*sin(alphaAB-pi./2.0).*cos(q2)+LB.*ddq2.*sin(alphaAB-pi./2.0).*sin(q2)).*(x+aB.*sin(alphaAB)-eB.*sin(alphaAB)+LB.*cos(q2).*sin(alphaAB)))./lB+((-ddx+LB.*dq2.^2.*cos(q2).*cos(alphaAB-pi./2.0)+LB.*ddq2.*sin(q2).*cos(alphaAB-pi./2.0)).*(y+aB.*cos(alphaAB)-eB.*cos(alphaAB)+LB.*cos(alphaAB).*cos(q2)))./lB))./(lB.*2.0)+(IlBxy.*(((ddz+LB.*ddq2.*sin(pi./2.0).*cos(q2)-LB.*dq2.^2.*sin(pi./2.0).*sin(q2)).*(x+aB.*sin(alphaAB)-eB.*sin(alphaAB)+LB.*cos(q2).*sin(alphaAB)))./lB-((dz+LB.*dq2.*cos(q2)).*(dx-LB.*dq2.*sin(q2).*cos(alphaAB-pi./2.0)))./lB+((dx-LB.*dq2.*sin(alphaAB).*sin(q2)).*(dz+LB.*dq2.*sin(pi./2.0).*cos(q2)))./lB+((z+LB.*sin(q2)).*(-ddx+LB.*dq2.^2.*cos(q2).*cos(alphaAB-pi./2.0)+LB.*ddq2.*sin(q2).*cos(alphaAB-pi./2.0)))./lB))./(lB.*2.0)).*2.0+1.0./lC.^2.*(z+LC.*sin(q3)).*((IlCxx.*(((dz+LC.*dq3.*cos(q3)).*(dy+LC.*dq3.*sin(alphaAC-pi./2.0).*sin(q3)))./lC-((dy-LC.*dq3.*cos(alphaAC).*sin(q3)).*(dz+LC.*dq3.*sin(pi./2.0).*cos(q3)))./lC+((z+LC.*sin(q3)).*(ddy+LC.*dq3.^2.*sin(alphaAC-pi./2.0).*cos(q3)+LC.*ddq3.*sin(alphaAC-pi./2.0).*sin(q3)))./lC-((ddz+LC.*ddq3.*sin(pi./2.0).*cos(q3)-LC.*dq3.^2.*sin(pi./2.0).*sin(q3)).*(y+aC.*cos(alphaAC)-eC.*cos(alphaAC)+LC.*cos(alphaAC).*cos(q3)))./lC))./(lC.*2.0)-(IlCxz.*(-((dy-LC.*dq3.*cos(alphaAC).*sin(q3)).*(dx-LC.*dq3.*sin(q3).*cos(alphaAC-pi./2.0)))./lC+((dx-LC.*dq3.*sin(alphaAC).*sin(q3)).*(dy+LC.*dq3.*sin(alphaAC-pi./2.0).*sin(q3)))./lC+((ddy+LC.*dq3.^2.*sin(alphaAC-pi./2.0).*cos(q3)+LC.*ddq3.*sin(alphaAC-pi./2.0).*sin(q3)).*(x+aC.*sin(alphaAC)-eC.*sin(alphaAC)+LC.*cos(q3).*sin(alphaAC)))./lC+((-ddx+LC.*dq3.^2.*cos(q3).*cos(alphaAC-pi./2.0)+LC.*ddq3.*sin(q3).*cos(alphaAC-pi./2.0)).*(y+aC.*cos(alphaAC)-eC.*cos(alphaAC)+LC.*cos(alphaAC).*cos(q3)))./lC))./(lC.*2.0)+(IlCxy.*(((ddz+LC.*ddq3.*sin(pi./2.0).*cos(q3)-LC.*dq3.^2.*sin(pi./2.0).*sin(q3)).*(x+aC.*sin(alphaAC)-eC.*sin(alphaAC)+LC.*cos(q3).*sin(alphaAC)))./lC-((dz+LC.*dq3.*cos(q3)).*(dx-LC.*dq3.*sin(q3).*cos(alphaAC-pi./2.0)))./lC+((dx-LC.*dq3.*sin(alphaAC).*sin(q3)).*(dz+LC.*dq3.*sin(pi./2.0).*cos(q3)))./lC+((z+LC.*sin(q3)).*(-ddx+LC.*dq3.^2.*cos(q3).*cos(alphaAC-pi./2.0)+LC.*ddq3.*sin(q3).*cos(alphaAC-pi./2.0)))./lC))./(lC.*2.0)).*2.0+(((IlAxz.*1.0./lA.^2.*(dx-LA.*dq1.*sin(q1).*cos(alphaAA-pi./2.0)))./2.0-(IlAxx.*1.0./lA.^2.*(dz+LA.*dq1.*sin(pi./2.0).*cos(q1)))./2.0).*(((dz+LA.*dq1.*sin(pi./2.0).*cos(q1)).*(y+aA.*cos(alphaAA)-eA.*cos(alphaAA)+LA.*cos(alphaAA).*cos(q1)))./lA-((z+LA.*sin(q1)).*(dy+LA.*dq1.*sin(alphaAA-pi./2.0).*sin(q1)))./lA).*2.0)./lA+(((IlBxz.*1.0./lB.^2.*(dx-LB.*dq2.*sin(q2).*cos(alphaAB-pi./2.0)))./2.0-(IlBxx.*1.0./lB.^2.*(dz+LB.*dq2.*sin(pi./2.0).*cos(q2)))./2.0).*(((dz+LB.*dq2.*sin(pi./2.0).*cos(q2)).*(y+aB.*cos(alphaAB)-eB.*cos(alphaAB)+LB.*cos(alphaAB).*cos(q2)))./lB-((z+LB.*sin(q2)).*(dy+LB.*dq2.*sin(alphaAB-pi./2.0).*sin(q2)))./lB).*2.0)./lB;ddz.*mTCP-g.*mTCP-g.*mlA-g.*mlB-g.*mlC+(mlA.*(ddz./2.0-(LA.*ddq1.*sin(pi./2.0).*cos(q1))./2.0+(LA.*dq1.^2.*sin(pi./2.0).*sin(q1))./2.0))./2.0+mlA.*(ddz./4.0-(LA.*ddq1.*sin(pi./2.0).*cos(q1))./4.0+(LA.*dq1.^2.*sin(pi./2.0).*sin(q1))./4.0)+(mlB.*(ddz./2.0-(LB.*ddq2.*sin(pi./2.0).*cos(q2))./2.0+(LB.*dq2.^2.*sin(pi./2.0).*sin(q2))./2.0))./2.0+mlB.*(ddz./4.0-(LB.*ddq2.*sin(pi./2.0).*cos(q2))./4.0+(LB.*dq2.^2.*sin(pi./2.0).*sin(q2))./4.0)+(mlC.*(ddz./2.0-(LC.*ddq3.*sin(pi./2.0).*cos(q3))./2.0+(LC.*dq3.^2.*sin(pi./2.0).*sin(q3))./2.0))./2.0+mlC.*(ddz./4.0-(LC.*ddq3.*sin(pi./2.0).*cos(q3))./4.0+(LC.*dq3.^2.*sin(pi./2.0).*sin(q3))./4.0)+1.0./lA.^2.*(dy-LA.*dq1.*cos(alphaAA).*sin(q1)).*((IlAxz.*(((dx-LA.*dq1.*sin(q1).*cos(alphaAA-pi./2.0)).*(y+aA.*cos(alphaAA)-eA.*cos(alphaAA)+LA.*cos(alphaAA).*cos(q1)))./lA-((dy+LA.*dq1.*sin(alphaAA-pi./2.0).*sin(q1)).*(x+aA.*sin(alphaAA)-eA.*sin(alphaAA)+LA.*cos(q1).*sin(alphaAA)))./lA).*(-1.0./2.0))./lA+(IlAxx.*(((dz+LA.*dq1.*sin(pi./2.0).*cos(q1)).*(y+aA.*cos(alphaAA)-eA.*cos(alphaAA)+LA.*cos(alphaAA).*cos(q1)))./lA-((z+LA.*sin(q1)).*(dy+LA.*dq1.*sin(alphaAA-pi./2.0).*sin(q1)))./lA))./(lA.*2.0)+(IlAxy.*(((z+LA.*sin(q1)).*(dx-LA.*dq1.*sin(q1).*cos(alphaAA-pi./2.0)))./lA-((dz+LA.*dq1.*sin(pi./2.0).*cos(q1)).*(x+aA.*sin(alphaAA)-eA.*sin(alphaAA)+LA.*cos(q1).*sin(alphaAA)))./lA))./(lA.*2.0)).*2.0+1.0./lB.^2.*(dy-LB.*dq2.*cos(alphaAB).*sin(q2)).*((IlBxz.*(((dx-LB.*dq2.*sin(q2).*cos(alphaAB-pi./2.0)).*(y+aB.*cos(alphaAB)-eB.*cos(alphaAB)+LB.*cos(alphaAB).*cos(q2)))./lB-((dy+LB.*dq2.*sin(alphaAB-pi./2.0).*sin(q2)).*(x+aB.*sin(alphaAB)-eB.*sin(alphaAB)+LB.*cos(q2).*sin(alphaAB)))./lB).*(-1.0./2.0))./lB+(IlBxx.*(((dz+LB.*dq2.*sin(pi./2.0).*cos(q2)).*(y+aB.*cos(alphaAB)-eB.*cos(alphaAB)+LB.*cos(alphaAB).*cos(q2)))./lB-((z+LB.*sin(q2)).*(dy+LB.*dq2.*sin(alphaAB-pi./2.0).*sin(q2)))./lB))./(lB.*2.0)+(IlBxy.*(((z+LB.*sin(q2)).*(dx-LB.*dq2.*sin(q2).*cos(alphaAB-pi./2.0)))./lB-((dz+LB.*dq2.*sin(pi./2.0).*cos(q2)).*(x+aB.*sin(alphaAB)-eB.*sin(alphaAB)+LB.*cos(q2).*sin(alphaAB)))./lB))./(lB.*2.0)).*2.0+1.0./lC.^2.*(dy-LC.*dq3.*cos(alphaAC).*sin(q3)).*((IlCxz.*(((dx-LC.*dq3.*sin(q3).*cos(alphaAC-pi./2.0)).*(y+aC.*cos(alphaAC)-eC.*cos(alphaAC)+LC.*cos(alphaAC).*cos(q3)))./lC-((dy+LC.*dq3.*sin(alphaAC-pi./2.0).*sin(q3)).*(x+aC.*sin(alphaAC)-eC.*sin(alphaAC)+LC.*cos(q3).*sin(alphaAC)))./lC).*(-1.0./2.0))./lC+(IlCxx.*(((dz+LC.*dq3.*sin(pi./2.0).*cos(q3)).*(y+aC.*cos(alphaAC)-eC.*cos(alphaAC)+LC.*cos(alphaAC).*cos(q3)))./lC-((z+LC.*sin(q3)).*(dy+LC.*dq3.*sin(alphaAC-pi./2.0).*sin(q3)))./lC))./(lC.*2.0)+(IlCxy.*(((z+LC.*sin(q3)).*(dx-LC.*dq3.*sin(q3).*cos(alphaAC-pi./2.0)))./lC-((dz+LC.*dq3.*sin(pi./2.0).*cos(q3)).*(x+aC.*sin(alphaAC)-eC.*sin(alphaAC)+LC.*cos(q3).*sin(alphaAC)))./lC))./(lC.*2.0)).*2.0-1.0./lA.^2.*(dx-LA.*dq1.*sin(alphaAA).*sin(q1)).*((IlAyz.*(((dx-LA.*dq1.*sin(q1).*cos(alphaAA-pi./2.0)).*(y+aA.*cos(alphaAA)-eA.*cos(alphaAA)+LA.*cos(alphaAA).*cos(q1)))./lA-((dy+LA.*dq1.*sin(alphaAA-pi./2.0).*sin(q1)).*(x+aA.*sin(alphaAA)-eA.*sin(alphaAA)+LA.*cos(q1).*sin(alphaAA)))./lA).*(-1.0./2.0))./lA+(IlAxy.*(((dz+LA.*dq1.*sin(pi./2.0).*cos(q1)).*(y+aA.*cos(alphaAA)-eA.*cos(alphaAA)+LA.*cos(alphaAA).*cos(q1)))./lA-((z+LA.*sin(q1)).*(dy+LA.*dq1.*sin(alphaAA-pi./2.0).*sin(q1)))./lA))./(lA.*2.0)+(IlAyy.*(((z+LA.*sin(q1)).*(dx-LA.*dq1.*sin(q1).*cos(alphaAA-pi./2.0)))./lA-((dz+LA.*dq1.*sin(pi./2.0).*cos(q1)).*(x+aA.*sin(alphaAA)-eA.*sin(alphaAA)+LA.*cos(q1).*sin(alphaAA)))./lA))./(lA.*2.0)).*2.0-1.0./lB.^2.*(dx-LB.*dq2.*sin(alphaAB).*sin(q2)).*((IlByz.*(((dx-LB.*dq2.*sin(q2).*cos(alphaAB-pi./2.0)).*(y+aB.*cos(alphaAB)-eB.*cos(alphaAB)+LB.*cos(alphaAB).*cos(q2)))./lB-((dy+LB.*dq2.*sin(alphaAB-pi./2.0).*sin(q2)).*(x+aB.*sin(alphaAB)-eB.*sin(alphaAB)+LB.*cos(q2).*sin(alphaAB)))./lB).*(-1.0./2.0))./lB+(IlBxy.*(((dz+LB.*dq2.*sin(pi./2.0).*cos(q2)).*(y+aB.*cos(alphaAB)-eB.*cos(alphaAB)+LB.*cos(alphaAB).*cos(q2)))./lB-((z+LB.*sin(q2)).*(dy+LB.*dq2.*sin(alphaAB-pi./2.0).*sin(q2)))./lB))./(lB.*2.0)+(IlByy.*(((z+LB.*sin(q2)).*(dx-LB.*dq2.*sin(q2).*cos(alphaAB-pi./2.0)))./lB-((dz+LB.*dq2.*sin(pi./2.0).*cos(q2)).*(x+aB.*sin(alphaAB)-eB.*sin(alphaAB)+LB.*cos(q2).*sin(alphaAB)))./lB))./(lB.*2.0)).*2.0-1.0./lC.^2.*(dx-LC.*dq3.*sin(alphaAC).*sin(q3)).*((IlCyz.*(((dx-LC.*dq3.*sin(q3).*cos(alphaAC-pi./2.0)).*(y+aC.*cos(alphaAC)-eC.*cos(alphaAC)+LC.*cos(alphaAC).*cos(q3)))./lC-((dy+LC.*dq3.*sin(alphaAC-pi./2.0).*sin(q3)).*(x+aC.*sin(alphaAC)-eC.*sin(alphaAC)+LC.*cos(q3).*sin(alphaAC)))./lC).*(-1.0./2.0))./lC+(IlCxy.*(((dz+LC.*dq3.*sin(pi./2.0).*cos(q3)).*(y+aC.*cos(alphaAC)-eC.*cos(alphaAC)+LC.*cos(alphaAC).*cos(q3)))./lC-((z+LC.*sin(q3)).*(dy+LC.*dq3.*sin(alphaAC-pi./2.0).*sin(q3)))./lC))./(lC.*2.0)+(IlCyy.*(((z+LC.*sin(q3)).*(dx-LC.*dq3.*sin(q3).*cos(alphaAC-pi./2.0)))./lC-((dz+LC.*dq3.*sin(pi./2.0).*cos(q3)).*(x+aC.*sin(alphaAC)-eC.*sin(alphaAC)+LC.*cos(q3).*sin(alphaAC)))./lC))./(lC.*2.0)).*2.0+(((IlAyz.*1.0./lA.^2.*(dx-LA.*dq1.*sin(alphaAA).*sin(q1)))./2.0-(IlAxz.*1.0./lA.^2.*(dy-LA.*dq1.*cos(alphaAA).*sin(q1)))./2.0).*(((dx-LA.*dq1.*sin(q1).*cos(alphaAA-pi./2.0)).*(y+aA.*cos(alphaAA)-eA.*cos(alphaAA)+LA.*cos(alphaAA).*cos(q1)))./lA-((dy+LA.*dq1.*sin(alphaAA-pi./2.0).*sin(q1)).*(x+aA.*sin(alphaAA)-eA.*sin(alphaAA)+LA.*cos(q1).*sin(alphaAA)))./lA).*2.0)./lA+(((IlByz.*1.0./lB.^2.*(dx-LB.*dq2.*sin(alphaAB).*sin(q2)))./2.0-(IlBxz.*1.0./lB.^2.*(dy-LB.*dq2.*cos(alphaAB).*sin(q2)))./2.0).*(((dx-LB.*dq2.*sin(q2).*cos(alphaAB-pi./2.0)).*(y+aB.*cos(alphaAB)-eB.*cos(alphaAB)+LB.*cos(alphaAB).*cos(q2)))./lB-((dy+LB.*dq2.*sin(alphaAB-pi./2.0).*sin(q2)).*(x+aB.*sin(alphaAB)-eB.*sin(alphaAB)+LB.*cos(q2).*sin(alphaAB)))./lB).*2.0)./lB+(((IlCyz.*1.0./lC.^2.*(dx-LC.*dq3.*sin(alphaAC).*sin(q3)))./2.0-(IlCxz.*1.0./lC.^2.*(dy-LC.*dq3.*cos(alphaAC).*sin(q3)))./2.0).*(((dx-LC.*dq3.*sin(q3).*cos(alphaAC-pi./2.0)).*(y+aC.*cos(alphaAC)-eC.*cos(alphaAC)+LC.*cos(alphaAC).*cos(q3)))./lC-((dy+LC.*dq3.*sin(alphaAC-pi./2.0).*sin(q3)).*(x+aC.*sin(alphaAC)-eC.*sin(alphaAC)+LC.*cos(q3).*sin(alphaAC)))./lC).*2.0)./lC-1.0./lA.^2.*(dx-LA.*dq1.*sin(q1).*cos(alphaAA-pi./2.0)).*((IlAyz.*(((dx-LA.*dq1.*sin(q1).*cos(alphaAA-pi./2.0)).*(y+aA.*cos(alphaAA)-eA.*cos(alphaAA)+LA.*cos(alphaAA).*cos(q1)))./lA-((dy+LA.*dq1.*sin(alphaAA-pi./2.0).*sin(q1)).*(x+aA.*sin(alphaAA)-eA.*sin(alphaAA)+LA.*cos(q1).*sin(alphaAA)))./lA).*(-1.0./2.0))./lA+(IlAxy.*(((dz+LA.*dq1.*sin(pi./2.0).*cos(q1)).*(y+aA.*cos(alphaAA)-eA.*cos(alphaAA)+LA.*cos(alphaAA).*cos(q1)))./lA-((z+LA.*sin(q1)).*(dy+LA.*dq1.*sin(alphaAA-pi./2.0).*sin(q1)))./lA))./(lA.*2.0)+(IlAyy.*(((z+LA.*sin(q1)).*(dx-LA.*dq1.*sin(q1).*cos(alphaAA-pi./2.0)))./lA-((dz+LA.*dq1.*sin(pi./2.0).*cos(q1)).*(x+aA.*sin(alphaAA)-eA.*sin(alphaAA)+LA.*cos(q1).*sin(alphaAA)))./lA))./(lA.*2.0)).*2.0-1.0./lB.^2.*(dx-LB.*dq2.*sin(q2).*cos(alphaAB-pi./2.0)).*((IlByz.*(((dx-LB.*dq2.*sin(q2).*cos(alphaAB-pi./2.0)).*(y+aB.*cos(alphaAB)-eB.*cos(alphaAB)+LB.*cos(alphaAB).*cos(q2)))./lB-((dy+LB.*dq2.*sin(alphaAB-pi./2.0).*sin(q2)).*(x+aB.*sin(alphaAB)-eB.*sin(alphaAB)+LB.*cos(q2).*sin(alphaAB)))./lB).*(-1.0./2.0))./lB+(IlBxy.*(((dz+LB.*dq2.*sin(pi./2.0).*cos(q2)).*(y+aB.*cos(alphaAB)-eB.*cos(alphaAB)+LB.*cos(alphaAB).*cos(q2)))./lB-((z+LB.*sin(q2)).*(dy+LB.*dq2.*sin(alphaAB-pi./2.0).*sin(q2)))./lB))./(lB.*2.0)+(IlByy.*(((z+LB.*sin(q2)).*(dx-LB.*dq2.*sin(q2).*cos(alphaAB-pi./2.0)))./lB-((dz+LB.*dq2.*sin(pi./2.0).*cos(q2)).*(x+aB.*sin(alphaAB)-eB.*sin(alphaAB)+LB.*cos(q2).*sin(alphaAB)))./lB))./(lB.*2.0)).*2.0-1.0./lC.^2.*(dx-LC.*dq3.*sin(q3).*cos(alphaAC-pi./2.0)).*((IlCyz.*(((dx-LC.*dq3.*sin(q3).*cos(alphaAC-pi./2.0)).*(y+aC.*cos(alphaAC)-eC.*cos(alphaAC)+LC.*cos(alphaAC).*cos(q3)))./lC-((dy+LC.*dq3.*sin(alphaAC-pi./2.0).*sin(q3)).*(x+aC.*sin(alphaAC)-eC.*sin(alphaAC)+LC.*cos(q3).*sin(alphaAC)))./lC).*(-1.0./2.0))./lC+(IlCxy.*(((dz+LC.*dq3.*sin(pi./2.0).*cos(q3)).*(y+aC.*cos(alphaAC)-eC.*cos(alphaAC)+LC.*cos(alphaAC).*cos(q3)))./lC-((z+LC.*sin(q3)).*(dy+LC.*dq3.*sin(alphaAC-pi./2.0).*sin(q3)))./lC))./(lC.*2.0)+(IlCyy.*(((z+LC.*sin(q3)).*(dx-LC.*dq3.*sin(q3).*cos(alphaAC-pi./2.0)))./lC-((dz+LC.*dq3.*sin(pi./2.0).*cos(q3)).*(x+aC.*sin(alphaAC)-eC.*sin(alphaAC)+LC.*cos(q3).*sin(alphaAC)))./lC))./(lC.*2.0)).*2.0+(((IlAxz.*1.0./lA.^2.*(y+aA.*cos(alphaAA)-eA.*cos(alphaAA)+LA.*cos(alphaAA).*cos(q1)))./2.0-(IlAyz.*1.0./lA.^2.*(x+aA.*sin(alphaAA)-eA.*sin(alphaAA)+LA.*cos(q1).*sin(alphaAA)))./2.0).*(-((dy-LA.*dq1.*cos(alphaAA).*sin(q1)).*(dx-LA.*dq1.*sin(q1).*cos(alphaAA-pi./2.0)))./lA+((dx-LA.*dq1.*sin(alphaAA).*sin(q1)).*(dy+LA.*dq1.*sin(alphaAA-pi./2.0).*sin(q1)))./lA+((ddy+LA.*dq1.^2.*sin(alphaAA-pi./2.0).*cos(q1)+LA.*ddq1.*sin(alphaAA-pi./2.0).*sin(q1)).*(x+aA.*sin(alphaAA)-eA.*sin(alphaAA)+LA.*cos(q1).*sin(alphaAA)))./lA+((-ddx+LA.*dq1.^2.*cos(q1).*cos(alphaAA-pi./2.0)+LA.*ddq1.*sin(q1).*cos(alphaAA-pi./2.0)).*(y+aA.*cos(alphaAA)-eA.*cos(alphaAA)+LA.*cos(alphaAA).*cos(q1)))./lA).*2.0)./lA+(((IlBxz.*1.0./lB.^2.*(y+aB.*cos(alphaAB)-eB.*cos(alphaAB)+LB.*cos(alphaAB).*cos(q2)))./2.0-(IlByz.*1.0./lB.^2.*(x+aB.*sin(alphaAB)-eB.*sin(alphaAB)+LB.*cos(q2).*sin(alphaAB)))./2.0).*(-((dy-LB.*dq2.*cos(alphaAB).*sin(q2)).*(dx-LB.*dq2.*sin(q2).*cos(alphaAB-pi./2.0)))./lB+((dx-LB.*dq2.*sin(alphaAB).*sin(q2)).*(dy+LB.*dq2.*sin(alphaAB-pi./2.0).*sin(q2)))./lB+((ddy+LB.*dq2.^2.*sin(alphaAB-pi./2.0).*cos(q2)+LB.*ddq2.*sin(alphaAB-pi./2.0).*sin(q2)).*(x+aB.*sin(alphaAB)-eB.*sin(alphaAB)+LB.*cos(q2).*sin(alphaAB)))./lB+((-ddx+LB.*dq2.^2.*cos(q2).*cos(alphaAB-pi./2.0)+LB.*ddq2.*sin(q2).*cos(alphaAB-pi./2.0)).*(y+aB.*cos(alphaAB)-eB.*cos(alphaAB)+LB.*cos(alphaAB).*cos(q2)))./lB).*2.0)./lB+(((IlCxz.*1.0./lC.^2.*(y+aC.*cos(alphaAC)-eC.*cos(alphaAC)+LC.*cos(alphaAC).*cos(q3)))./2.0-(IlCyz.*1.0./lC.^2.*(x+aC.*sin(alphaAC)-eC.*sin(alphaAC)+LC.*cos(q3).*sin(alphaAC)))./2.0).*(-((dy-LC.*dq3.*cos(alphaAC).*sin(q3)).*(dx-LC.*dq3.*sin(q3).*cos(alphaAC-pi./2.0)))./lC+((dx-LC.*dq3.*sin(alphaAC).*sin(q3)).*(dy+LC.*dq3.*sin(alphaAC-pi./2.0).*sin(q3)))./lC+((ddy+LC.*dq3.^2.*sin(alphaAC-pi./2.0).*cos(q3)+LC.*ddq3.*sin(alphaAC-pi./2.0).*sin(q3)).*(x+aC.*sin(alphaAC)-eC.*sin(alphaAC)+LC.*cos(q3).*sin(alphaAC)))./lC+((-ddx+LC.*dq3.^2.*cos(q3).*cos(alphaAC-pi./2.0)+LC.*ddq3.*sin(q3).*cos(alphaAC-pi./2.0)).*(y+aC.*cos(alphaAC)-eC.*cos(alphaAC)+LC.*cos(alphaAC).*cos(q3)))./lC).*2.0)./lC+1.0./lA.^2.*(dy+LA.*dq1.*sin(alphaAA-pi./2.0).*sin(q1)).*((IlAxz.*(((dx-LA.*dq1.*sin(q1).*cos(alphaAA-pi./2.0)).*(y+aA.*cos(alphaAA)-eA.*cos(alphaAA)+LA.*cos(alphaAA).*cos(q1)))./lA-((dy+LA.*dq1.*sin(alphaAA-pi./2.0).*sin(q1)).*(x+aA.*sin(alphaAA)-eA.*sin(alphaAA)+LA.*cos(q1).*sin(alphaAA)))./lA).*(-1.0./2.0))./lA+(IlAxx.*(((dz+LA.*dq1.*sin(pi./2.0).*cos(q1)).*(y+aA.*cos(alphaAA)-eA.*cos(alphaAA)+LA.*cos(alphaAA).*cos(q1)))./lA-((z+LA.*sin(q1)).*(dy+LA.*dq1.*sin(alphaAA-pi./2.0).*sin(q1)))./lA))./(lA.*2.0)+(IlAxy.*(((z+LA.*sin(q1)).*(dx-LA.*dq1.*sin(q1).*cos(alphaAA-pi./2.0)))./lA-((dz+LA.*dq1.*sin(pi./2.0).*cos(q1)).*(x+aA.*sin(alphaAA)-eA.*sin(alphaAA)+LA.*cos(q1).*sin(alphaAA)))./lA))./(lA.*2.0)).*2.0+1.0./lB.^2.*(dy+LB.*dq2.*sin(alphaAB-pi./2.0).*sin(q2)).*((IlBxz.*(((dx-LB.*dq2.*sin(q2).*cos(alphaAB-pi./2.0)).*(y+aB.*cos(alphaAB)-eB.*cos(alphaAB)+LB.*cos(alphaAB).*cos(q2)))./lB-((dy+LB.*dq2.*sin(alphaAB-pi./2.0).*sin(q2)).*(x+aB.*sin(alphaAB)-eB.*sin(alphaAB)+LB.*cos(q2).*sin(alphaAB)))./lB).*(-1.0./2.0))./lB+(IlBxx.*(((dz+LB.*dq2.*sin(pi./2.0).*cos(q2)).*(y+aB.*cos(alphaAB)-eB.*cos(alphaAB)+LB.*cos(alphaAB).*cos(q2)))./lB-((z+LB.*sin(q2)).*(dy+LB.*dq2.*sin(alphaAB-pi./2.0).*sin(q2)))./lB))./(lB.*2.0)+(IlBxy.*(((z+LB.*sin(q2)).*(dx-LB.*dq2.*sin(q2).*cos(alphaAB-pi./2.0)))./lB-((dz+LB.*dq2.*sin(pi./2.0).*cos(q2)).*(x+aB.*sin(alphaAB)-eB.*sin(alphaAB)+LB.*cos(q2).*sin(alphaAB)))./lB))./(lB.*2.0)).*2.0+1.0./lC.^2.*(dy+LC.*dq3.*sin(alphaAC-pi./2.0).*sin(q3)).*((IlCxz.*(((dx-LC.*dq3.*sin(q3).*cos(alphaAC-pi./2.0)).*(y+aC.*cos(alphaAC)-eC.*cos(alphaAC)+LC.*cos(alphaAC).*cos(q3)))./lC-((dy+LC.*dq3.*sin(alphaAC-pi./2.0).*sin(q3)).*(x+aC.*sin(alphaAC)-eC.*sin(alphaAC)+LC.*cos(q3).*sin(alphaAC)))./lC).*(-1.0./2.0))./lC+(IlCxx.*(((dz+LC.*dq3.*sin(pi./2.0).*cos(q3)).*(y+aC.*cos(alphaAC)-eC.*cos(alphaAC)+LC.*cos(alphaAC).*cos(q3)))./lC-((z+LC.*sin(q3)).*(dy+LC.*dq3.*sin(alphaAC-pi./2.0).*sin(q3)))./lC))./(lC.*2.0)+(IlCxy.*(((z+LC.*sin(q3)).*(dx-LC.*dq3.*sin(q3).*cos(alphaAC-pi./2.0)))./lC-((dz+LC.*dq3.*sin(pi./2.0).*cos(q3)).*(x+aC.*sin(alphaAC)-eC.*sin(alphaAC)+LC.*cos(q3).*sin(alphaAC)))./lC))./(lC.*2.0)).*2.0-(((IlAxy.*1.0./lA.^2.*(y+aA.*cos(alphaAA)-eA.*cos(alphaAA)+LA.*cos(alphaAA).*cos(q1)))./2.0-(IlAyy.*1.0./lA.^2.*(x+aA.*sin(alphaAA)-eA.*sin(alphaAA)+LA.*cos(q1).*sin(alphaAA)))./2.0).*(((ddz+LA.*ddq1.*sin(pi./2.0).*cos(q1)-LA.*dq1.^2.*sin(pi./2.0).*sin(q1)).*(x+aA.*sin(alphaAA)-eA.*sin(alphaAA)+LA.*cos(q1).*sin(alphaAA)))./lA-((dz+LA.*dq1.*cos(q1)).*(dx-LA.*dq1.*sin(q1).*cos(alphaAA-pi./2.0)))./lA+((dx-LA.*dq1.*sin(alphaAA).*sin(q1)).*(dz+LA.*dq1.*sin(pi./2.0).*cos(q1)))./lA+((z+LA.*sin(q1)).*(-ddx+LA.*dq1.^2.*cos(q1).*cos(alphaAA-pi./2.0)+LA.*ddq1.*sin(q1).*cos(alphaAA-pi./2.0)))./lA).*2.0)./lA-(((IlBxy.*1.0./lB.^2.*(y+aB.*cos(alphaAB)-eB.*cos(alphaAB)+LB.*cos(alphaAB).*cos(q2)))./2.0-(IlByy.*1.0./lB.^2.*(x+aB.*sin(alphaAB)-eB.*sin(alphaAB)+LB.*cos(q2).*sin(alphaAB)))./2.0).*(((ddz+LB.*ddq2.*sin(pi./2.0).*cos(q2)-LB.*dq2.^2.*sin(pi./2.0).*sin(q2)).*(x+aB.*sin(alphaAB)-eB.*sin(alphaAB)+LB.*cos(q2).*sin(alphaAB)))./lB-((dz+LB.*dq2.*cos(q2)).*(dx-LB.*dq2.*sin(q2).*cos(alphaAB-pi./2.0)))./lB+((dx-LB.*dq2.*sin(alphaAB).*sin(q2)).*(dz+LB.*dq2.*sin(pi./2.0).*cos(q2)))./lB+((z+LB.*sin(q2)).*(-ddx+LB.*dq2.^2.*cos(q2).*cos(alphaAB-pi./2.0)+LB.*ddq2.*sin(q2).*cos(alphaAB-pi./2.0)))./lB).*2.0)./lB-(((IlCxy.*1.0./lC.^2.*(y+aC.*cos(alphaAC)-eC.*cos(alphaAC)+LC.*cos(alphaAC).*cos(q3)))./2.0-(IlCyy.*1.0./lC.^2.*(x+aC.*sin(alphaAC)-eC.*sin(alphaAC)+LC.*cos(q3).*sin(alphaAC)))./2.0).*(((ddz+LC.*ddq3.*sin(pi./2.0).*cos(q3)-LC.*dq3.^2.*sin(pi./2.0).*sin(q3)).*(x+aC.*sin(alphaAC)-eC.*sin(alphaAC)+LC.*cos(q3).*sin(alphaAC)))./lC-((dz+LC.*dq3.*cos(q3)).*(dx-LC.*dq3.*sin(q3).*cos(alphaAC-pi./2.0)))./lC+((dx-LC.*dq3.*sin(alphaAC).*sin(q3)).*(dz+LC.*dq3.*sin(pi./2.0).*cos(q3)))./lC+((z+LC.*sin(q3)).*(-ddx+LC.*dq3.^2.*cos(q3).*cos(alphaAC-pi./2.0)+LC.*ddq3.*sin(q3).*cos(alphaAC-pi./2.0)))./lC).*2.0)./lC-(((IlAxy.*1.0./lA.^2.*(dx-LA.*dq1.*sin(alphaAA).*sin(q1)))./2.0-(IlAxx.*1.0./lA.^2.*(dy-LA.*dq1.*cos(alphaAA).*sin(q1)))./2.0).*(((dz+LA.*dq1.*sin(pi./2.0).*cos(q1)).*(y+aA.*cos(alphaAA)-eA.*cos(alphaAA)+LA.*cos(alphaAA).*cos(q1)))./lA-((z+LA.*sin(q1)).*(dy+LA.*dq1.*sin(alphaAA-pi./2.0).*sin(q1)))./lA).*2.0)./lA-(((IlBxy.*1.0./lB.^2.*(dx-LB.*dq2.*sin(alphaAB).*sin(q2)))./2.0-(IlBxx.*1.0./lB.^2.*(dy-LB.*dq2.*cos(alphaAB).*sin(q2)))./2.0).*(((dz+LB.*dq2.*sin(pi./2.0).*cos(q2)).*(y+aB.*cos(alphaAB)-eB.*cos(alphaAB)+LB.*cos(alphaAB).*cos(q2)))./lB-((z+LB.*sin(q2)).*(dy+LB.*dq2.*sin(alphaAB-pi./2.0).*sin(q2)))./lB).*2.0)./lB-(((IlCxy.*1.0./lC.^2.*(dx-LC.*dq3.*sin(alphaAC).*sin(q3)))./2.0-(IlCxx.*1.0./lC.^2.*(dy-LC.*dq3.*cos(alphaAC).*sin(q3)))./2.0).*(((dz+LC.*dq3.*sin(pi./2.0).*cos(q3)).*(y+aC.*cos(alphaAC)-eC.*cos(alphaAC)+LC.*cos(alphaAC).*cos(q3)))./lC-((z+LC.*sin(q3)).*(dy+LC.*dq3.*sin(alphaAC-pi./2.0).*sin(q3)))./lC).*2.0)./lC+((((dx-LA.*dq1.*sin(q1).*cos(alphaAA-pi./2.0)).*(y+aA.*cos(alphaAA)-eA.*cos(alphaAA)+LA.*cos(alphaAA).*cos(q1)))./lA-((dy+LA.*dq1.*sin(alphaAA-pi./2.0).*sin(q1)).*(x+aA.*sin(alphaAA)-eA.*sin(alphaAA)+LA.*cos(q1).*sin(alphaAA)))./lA).*((IlAyz.*1.0./lA.^2.*(dx-LA.*dq1.*sin(q1).*cos(alphaAA-pi./2.0)))./2.0-(IlAxz.*1.0./lA.^2.*(dy+LA.*dq1.*sin(alphaAA-pi./2.0).*sin(q1)))./2.0).*2.0)./lA+((((dx-LB.*dq2.*sin(q2).*cos(alphaAB-pi./2.0)).*(y+aB.*cos(alphaAB)-eB.*cos(alphaAB)+LB.*cos(alphaAB).*cos(q2)))./lB-((dy+LB.*dq2.*sin(alphaAB-pi./2.0).*sin(q2)).*(x+aB.*sin(alphaAB)-eB.*sin(alphaAB)+LB.*cos(q2).*sin(alphaAB)))./lB).*((IlByz.*1.0./lB.^2.*(dx-LB.*dq2.*sin(q2).*cos(alphaAB-pi./2.0)))./2.0-(IlBxz.*1.0./lB.^2.*(dy+LB.*dq2.*sin(alphaAB-pi./2.0).*sin(q2)))./2.0).*2.0)./lB+((((dx-LC.*dq3.*sin(q3).*cos(alphaAC-pi./2.0)).*(y+aC.*cos(alphaAC)-eC.*cos(alphaAC)+LC.*cos(alphaAC).*cos(q3)))./lC-((dy+LC.*dq3.*sin(alphaAC-pi./2.0).*sin(q3)).*(x+aC.*sin(alphaAC)-eC.*sin(alphaAC)+LC.*cos(q3).*sin(alphaAC)))./lC).*((IlCyz.*1.0./lC.^2.*(dx-LC.*dq3.*sin(q3).*cos(alphaAC-pi./2.0)))./2.0-(IlCxz.*1.0./lC.^2.*(dy+LC.*dq3.*sin(alphaAC-pi./2.0).*sin(q3)))./2.0).*2.0)./lC-((((z+LA.*sin(q1)).*(dx-LA.*dq1.*sin(q1).*cos(alphaAA-pi./2.0)))./lA-((dz+LA.*dq1.*sin(pi./2.0).*cos(q1)).*(x+aA.*sin(alphaAA)-eA.*sin(alphaAA)+LA.*cos(q1).*sin(alphaAA)))./lA).*((IlAyy.*1.0./lA.^2.*(dx-LA.*dq1.*sin(alphaAA).*sin(q1)))./2.0-(IlAxy.*1.0./lA.^2.*(dy-LA.*dq1.*cos(alphaAA).*sin(q1)))./2.0).*2.0)./lA-((((z+LB.*sin(q2)).*(dx-LB.*dq2.*sin(q2).*cos(alphaAB-pi./2.0)))./lB-((dz+LB.*dq2.*sin(pi./2.0).*cos(q2)).*(x+aB.*sin(alphaAB)-eB.*sin(alphaAB)+LB.*cos(q2).*sin(alphaAB)))./lB).*((IlByy.*1.0./lB.^2.*(dx-LB.*dq2.*sin(alphaAB).*sin(q2)))./2.0-(IlBxy.*1.0./lB.^2.*(dy-LB.*dq2.*cos(alphaAB).*sin(q2)))./2.0).*2.0)./lB-((((z+LC.*sin(q3)).*(dx-LC.*dq3.*sin(q3).*cos(alphaAC-pi./2.0)))./lC-((dz+LC.*dq3.*sin(pi./2.0).*cos(q3)).*(x+aC.*sin(alphaAC)-eC.*sin(alphaAC)+LC.*cos(q3).*sin(alphaAC)))./lC).*((IlCyy.*1.0./lC.^2.*(dx-LC.*dq3.*sin(alphaAC).*sin(q3)))./2.0-(IlCxy.*1.0./lC.^2.*(dy-LC.*dq3.*cos(alphaAC).*sin(q3)))./2.0).*2.0)./lC-1.0./lA.^2.*((IlAxx.*(((dz+LA.*dq1.*cos(q1)).*(dy+LA.*dq1.*sin(alphaAA-pi./2.0).*sin(q1)))./lA-((dy-LA.*dq1.*cos(alphaAA).*sin(q1)).*(dz+LA.*dq1.*sin(pi./2.0).*cos(q1)))./lA+((z+LA.*sin(q1)).*(ddy+LA.*dq1.^2.*sin(alphaAA-pi./2.0).*cos(q1)+LA.*ddq1.*sin(alphaAA-pi./2.0).*sin(q1)))./lA-((ddz+LA.*ddq1.*sin(pi./2.0).*cos(q1)-LA.*dq1.^2.*sin(pi./2.0).*sin(q1)).*(y+aA.*cos(alphaAA)-eA.*cos(alphaAA)+LA.*cos(alphaAA).*cos(q1)))./lA))./(lA.*2.0)-(IlAxz.*(-((dy-LA.*dq1.*cos(alphaAA).*sin(q1)).*(dx-LA.*dq1.*sin(q1).*cos(alphaAA-pi./2.0)))./lA+((dx-LA.*dq1.*sin(alphaAA).*sin(q1)).*(dy+LA.*dq1.*sin(alphaAA-pi./2.0).*sin(q1)))./lA+((ddy+LA.*dq1.^2.*sin(alphaAA-pi./2.0).*cos(q1)+LA.*ddq1.*sin(alphaAA-pi./2.0).*sin(q1)).*(x+aA.*sin(alphaAA)-eA.*sin(alphaAA)+LA.*cos(q1).*sin(alphaAA)))./lA+((-ddx+LA.*dq1.^2.*cos(q1).*cos(alphaAA-pi./2.0)+LA.*ddq1.*sin(q1).*cos(alphaAA-pi./2.0)).*(y+aA.*cos(alphaAA)-eA.*cos(alphaAA)+LA.*cos(alphaAA).*cos(q1)))./lA))./(lA.*2.0)+(IlAxy.*(((ddz+LA.*ddq1.*sin(pi./2.0).*cos(q1)-LA.*dq1.^2.*sin(pi./2.0).*sin(q1)).*(x+aA.*sin(alphaAA)-eA.*sin(alphaAA)+LA.*cos(q1).*sin(alphaAA)))./lA-((dz+LA.*dq1.*cos(q1)).*(dx-LA.*dq1.*sin(q1).*cos(alphaAA-pi./2.0)))./lA+((dx-LA.*dq1.*sin(alphaAA).*sin(q1)).*(dz+LA.*dq1.*sin(pi./2.0).*cos(q1)))./lA+((z+LA.*sin(q1)).*(-ddx+LA.*dq1.^2.*cos(q1).*cos(alphaAA-pi./2.0)+LA.*ddq1.*sin(q1).*cos(alphaAA-pi./2.0)))./lA))./(lA.*2.0)).*(y+aA.*cos(alphaAA)-eA.*cos(alphaAA)+LA.*cos(alphaAA).*cos(q1)).*2.0-1.0./lB.^2.*((IlBxx.*(((dz+LB.*dq2.*cos(q2)).*(dy+LB.*dq2.*sin(alphaAB-pi./2.0).*sin(q2)))./lB-((dy-LB.*dq2.*cos(alphaAB).*sin(q2)).*(dz+LB.*dq2.*sin(pi./2.0).*cos(q2)))./lB+((z+LB.*sin(q2)).*(ddy+LB.*dq2.^2.*sin(alphaAB-pi./2.0).*cos(q2)+LB.*ddq2.*sin(alphaAB-pi./2.0).*sin(q2)))./lB-((ddz+LB.*ddq2.*sin(pi./2.0).*cos(q2)-LB.*dq2.^2.*sin(pi./2.0).*sin(q2)).*(y+aB.*cos(alphaAB)-eB.*cos(alphaAB)+LB.*cos(alphaAB).*cos(q2)))./lB))./(lB.*2.0)-(IlBxz.*(-((dy-LB.*dq2.*cos(alphaAB).*sin(q2)).*(dx-LB.*dq2.*sin(q2).*cos(alphaAB-pi./2.0)))./lB+((dx-LB.*dq2.*sin(alphaAB).*sin(q2)).*(dy+LB.*dq2.*sin(alphaAB-pi./2.0).*sin(q2)))./lB+((ddy+LB.*dq2.^2.*sin(alphaAB-pi./2.0).*cos(q2)+LB.*ddq2.*sin(alphaAB-pi./2.0).*sin(q2)).*(x+aB.*sin(alphaAB)-eB.*sin(alphaAB)+LB.*cos(q2).*sin(alphaAB)))./lB+((-ddx+LB.*dq2.^2.*cos(q2).*cos(alphaAB-pi./2.0)+LB.*ddq2.*sin(q2).*cos(alphaAB-pi./2.0)).*(y+aB.*cos(alphaAB)-eB.*cos(alphaAB)+LB.*cos(alphaAB).*cos(q2)))./lB))./(lB.*2.0)+(IlBxy.*(((ddz+LB.*ddq2.*sin(pi./2.0).*cos(q2)-LB.*dq2.^2.*sin(pi./2.0).*sin(q2)).*(x+aB.*sin(alphaAB)-eB.*sin(alphaAB)+LB.*cos(q2).*sin(alphaAB)))./lB-((dz+LB.*dq2.*cos(q2)).*(dx-LB.*dq2.*sin(q2).*cos(alphaAB-pi./2.0)))./lB+((dx-LB.*dq2.*sin(alphaAB).*sin(q2)).*(dz+LB.*dq2.*sin(pi./2.0).*cos(q2)))./lB+((z+LB.*sin(q2)).*(-ddx+LB.*dq2.^2.*cos(q2).*cos(alphaAB-pi./2.0)+LB.*ddq2.*sin(q2).*cos(alphaAB-pi./2.0)))./lB))./(lB.*2.0)).*(y+aB.*cos(alphaAB)-eB.*cos(alphaAB)+LB.*cos(alphaAB).*cos(q2)).*2.0-1.0./lC.^2.*((IlCxx.*(((dz+LC.*dq3.*cos(q3)).*(dy+LC.*dq3.*sin(alphaAC-pi./2.0).*sin(q3)))./lC-((dy-LC.*dq3.*cos(alphaAC).*sin(q3)).*(dz+LC.*dq3.*sin(pi./2.0).*cos(q3)))./lC+((z+LC.*sin(q3)).*(ddy+LC.*dq3.^2.*sin(alphaAC-pi./2.0).*cos(q3)+LC.*ddq3.*sin(alphaAC-pi./2.0).*sin(q3)))./lC-((ddz+LC.*ddq3.*sin(pi./2.0).*cos(q3)-LC.*dq3.^2.*sin(pi./2.0).*sin(q3)).*(y+aC.*cos(alphaAC)-eC.*cos(alphaAC)+LC.*cos(alphaAC).*cos(q3)))./lC))./(lC.*2.0)-(IlCxz.*(-((dy-LC.*dq3.*cos(alphaAC).*sin(q3)).*(dx-LC.*dq3.*sin(q3).*cos(alphaAC-pi./2.0)))./lC+((dx-LC.*dq3.*sin(alphaAC).*sin(q3)).*(dy+LC.*dq3.*sin(alphaAC-pi./2.0).*sin(q3)))./lC+((ddy+LC.*dq3.^2.*sin(alphaAC-pi./2.0).*cos(q3)+LC.*ddq3.*sin(alphaAC-pi./2.0).*sin(q3)).*(x+aC.*sin(alphaAC)-eC.*sin(alphaAC)+LC.*cos(q3).*sin(alphaAC)))./lC+((-ddx+LC.*dq3.^2.*cos(q3).*cos(alphaAC-pi./2.0)+LC.*ddq3.*sin(q3).*cos(alphaAC-pi./2.0)).*(y+aC.*cos(alphaAC)-eC.*cos(alphaAC)+LC.*cos(alphaAC).*cos(q3)))./lC))./(lC.*2.0)+(IlCxy.*(((ddz+LC.*ddq3.*sin(pi./2.0).*cos(q3)-LC.*dq3.^2.*sin(pi./2.0).*sin(q3)).*(x+aC.*sin(alphaAC)-eC.*sin(alphaAC)+LC.*cos(q3).*sin(alphaAC)))./lC-((dz+LC.*dq3.*cos(q3)).*(dx-LC.*dq3.*sin(q3).*cos(alphaAC-pi./2.0)))./lC+((dx-LC.*dq3.*sin(alphaAC).*sin(q3)).*(dz+LC.*dq3.*sin(pi./2.0).*cos(q3)))./lC+((z+LC.*sin(q3)).*(-ddx+LC.*dq3.^2.*cos(q3).*cos(alphaAC-pi./2.0)+LC.*ddq3.*sin(q3).*cos(alphaAC-pi./2.0)))./lC))./(lC.*2.0)).*(y+aC.*cos(alphaAC)-eC.*cos(alphaAC)+LC.*cos(alphaAC).*cos(q3)).*2.0-(((IlAxy.*1.0./lA.^2.*(dx-LA.*dq1.*sin(q1).*cos(alphaAA-pi./2.0)))./2.0-(IlAxx.*1.0./lA.^2.*(dy+LA.*dq1.*sin(alphaAA-pi./2.0).*sin(q1)))./2.0).*(((dz+LA.*dq1.*sin(pi./2.0).*cos(q1)).*(y+aA.*cos(alphaAA)-eA.*cos(alphaAA)+LA.*cos(alphaAA).*cos(q1)))./lA-((z+LA.*sin(q1)).*(dy+LA.*dq1.*sin(alphaAA-pi./2.0).*sin(q1)))./lA).*2.0)./lA-(((IlBxy.*1.0./lB.^2.*(dx-LB.*dq2.*sin(q2).*cos(alphaAB-pi./2.0)))./2.0-(IlBxx.*1.0./lB.^2.*(dy+LB.*dq2.*sin(alphaAB-pi./2.0).*sin(q2)))./2.0).*(((dz+LB.*dq2.*sin(pi./2.0).*cos(q2)).*(y+aB.*cos(alphaAB)-eB.*cos(alphaAB)+LB.*cos(alphaAB).*cos(q2)))./lB-((z+LB.*sin(q2)).*(dy+LB.*dq2.*sin(alphaAB-pi./2.0).*sin(q2)))./lB).*2.0)./lB-(((IlCxy.*1.0./lC.^2.*(dx-LC.*dq3.*sin(q3).*cos(alphaAC-pi./2.0)))./2.0-(IlCxx.*1.0./lC.^2.*(dy+LC.*dq3.*sin(alphaAC-pi./2.0).*sin(q3)))./2.0).*(((dz+LC.*dq3.*sin(pi./2.0).*cos(q3)).*(y+aC.*cos(alphaAC)-eC.*cos(alphaAC)+LC.*cos(alphaAC).*cos(q3)))./lC-((z+LC.*sin(q3)).*(dy+LC.*dq3.*sin(alphaAC-pi./2.0).*sin(q3)))./lC).*2.0)./lC-((((z+LA.*sin(q1)).*(dx-LA.*dq1.*sin(q1).*cos(alphaAA-pi./2.0)))./lA-((dz+LA.*dq1.*sin(pi./2.0).*cos(q1)).*(x+aA.*sin(alphaAA)-eA.*sin(alphaAA)+LA.*cos(q1).*sin(alphaAA)))./lA).*((IlAyy.*1.0./lA.^2.*(dx-LA.*dq1.*sin(q1).*cos(alphaAA-pi./2.0)))./2.0-(IlAxy.*1.0./lA.^2.*(dy+LA.*dq1.*sin(alphaAA-pi./2.0).*sin(q1)))./2.0).*2.0)./lA-((((z+LB.*sin(q2)).*(dx-LB.*dq2.*sin(q2).*cos(alphaAB-pi./2.0)))./lB-((dz+LB.*dq2.*sin(pi./2.0).*cos(q2)).*(x+aB.*sin(alphaAB)-eB.*sin(alphaAB)+LB.*cos(q2).*sin(alphaAB)))./lB).*((IlByy.*1.0./lB.^2.*(dx-LB.*dq2.*sin(q2).*cos(alphaAB-pi./2.0)))./2.0-(IlBxy.*1.0./lB.^2.*(dy+LB.*dq2.*sin(alphaAB-pi./2.0).*sin(q2)))./2.0).*2.0)./lB-((((z+LC.*sin(q3)).*(dx-LC.*dq3.*sin(q3).*cos(alphaAC-pi./2.0)))./lC-((dz+LC.*dq3.*sin(pi./2.0).*cos(q3)).*(x+aC.*sin(alphaAC)-eC.*sin(alphaAC)+LC.*cos(q3).*sin(alphaAC)))./lC).*((IlCyy.*1.0./lC.^2.*(dx-LC.*dq3.*sin(q3).*cos(alphaAC-pi./2.0)))./2.0-(IlCxy.*1.0./lC.^2.*(dy+LC.*dq3.*sin(alphaAC-pi./2.0).*sin(q3)))./2.0).*2.0)./lC+1.0./lA.^2.*((IlAxy.*(((dz+LA.*dq1.*cos(q1)).*(dy+LA.*dq1.*sin(alphaAA-pi./2.0).*sin(q1)))./lA-((dy-LA.*dq1.*cos(alphaAA).*sin(q1)).*(dz+LA.*dq1.*sin(pi./2.0).*cos(q1)))./lA+((z+LA.*sin(q1)).*(ddy+LA.*dq1.^2.*sin(alphaAA-pi./2.0).*cos(q1)+LA.*ddq1.*sin(alphaAA-pi./2.0).*sin(q1)))./lA-((ddz+LA.*ddq1.*sin(pi./2.0).*cos(q1)-LA.*dq1.^2.*sin(pi./2.0).*sin(q1)).*(y+aA.*cos(alphaAA)-eA.*cos(alphaAA)+LA.*cos(alphaAA).*cos(q1)))./lA))./(lA.*2.0)-(IlAyz.*(-((dy-LA.*dq1.*cos(alphaAA).*sin(q1)).*(dx-LA.*dq1.*sin(q1).*cos(alphaAA-pi./2.0)))./lA+((dx-LA.*dq1.*sin(alphaAA).*sin(q1)).*(dy+LA.*dq1.*sin(alphaAA-pi./2.0).*sin(q1)))./lA+((ddy+LA.*dq1.^2.*sin(alphaAA-pi./2.0).*cos(q1)+LA.*ddq1.*sin(alphaAA-pi./2.0).*sin(q1)).*(x+aA.*sin(alphaAA)-eA.*sin(alphaAA)+LA.*cos(q1).*sin(alphaAA)))./lA+((-ddx+LA.*dq1.^2.*cos(q1).*cos(alphaAA-pi./2.0)+LA.*ddq1.*sin(q1).*cos(alphaAA-pi./2.0)).*(y+aA.*cos(alphaAA)-eA.*cos(alphaAA)+LA.*cos(alphaAA).*cos(q1)))./lA))./(lA.*2.0)+(IlAyy.*(((ddz+LA.*ddq1.*sin(pi./2.0).*cos(q1)-LA.*dq1.^2.*sin(pi./2.0).*sin(q1)).*(x+aA.*sin(alphaAA)-eA.*sin(alphaAA)+LA.*cos(q1).*sin(alphaAA)))./lA-((dz+LA.*dq1.*cos(q1)).*(dx-LA.*dq1.*sin(q1).*cos(alphaAA-pi./2.0)))./lA+((dx-LA.*dq1.*sin(alphaAA).*sin(q1)).*(dz+LA.*dq1.*sin(pi./2.0).*cos(q1)))./lA+((z+LA.*sin(q1)).*(-ddx+LA.*dq1.^2.*cos(q1).*cos(alphaAA-pi./2.0)+LA.*ddq1.*sin(q1).*cos(alphaAA-pi./2.0)))./lA))./(lA.*2.0)).*(x+aA.*sin(alphaAA)-eA.*sin(alphaAA)+LA.*cos(q1).*sin(alphaAA)).*2.0+1.0./lB.^2.*((IlBxy.*(((dz+LB.*dq2.*cos(q2)).*(dy+LB.*dq2.*sin(alphaAB-pi./2.0).*sin(q2)))./lB-((dy-LB.*dq2.*cos(alphaAB).*sin(q2)).*(dz+LB.*dq2.*sin(pi./2.0).*cos(q2)))./lB+((z+LB.*sin(q2)).*(ddy+LB.*dq2.^2.*sin(alphaAB-pi./2.0).*cos(q2)+LB.*ddq2.*sin(alphaAB-pi./2.0).*sin(q2)))./lB-((ddz+LB.*ddq2.*sin(pi./2.0).*cos(q2)-LB.*dq2.^2.*sin(pi./2.0).*sin(q2)).*(y+aB.*cos(alphaAB)-eB.*cos(alphaAB)+LB.*cos(alphaAB).*cos(q2)))./lB))./(lB.*2.0)-(IlByz.*(-((dy-LB.*dq2.*cos(alphaAB).*sin(q2)).*(dx-LB.*dq2.*sin(q2).*cos(alphaAB-pi./2.0)))./lB+((dx-LB.*dq2.*sin(alphaAB).*sin(q2)).*(dy+LB.*dq2.*sin(alphaAB-pi./2.0).*sin(q2)))./lB+((ddy+LB.*dq2.^2.*sin(alphaAB-pi./2.0).*cos(q2)+LB.*ddq2.*sin(alphaAB-pi./2.0).*sin(q2)).*(x+aB.*sin(alphaAB)-eB.*sin(alphaAB)+LB.*cos(q2).*sin(alphaAB)))./lB+((-ddx+LB.*dq2.^2.*cos(q2).*cos(alphaAB-pi./2.0)+LB.*ddq2.*sin(q2).*cos(alphaAB-pi./2.0)).*(y+aB.*cos(alphaAB)-eB.*cos(alphaAB)+LB.*cos(alphaAB).*cos(q2)))./lB))./(lB.*2.0)+(IlByy.*(((ddz+LB.*ddq2.*sin(pi./2.0).*cos(q2)-LB.*dq2.^2.*sin(pi./2.0).*sin(q2)).*(x+aB.*sin(alphaAB)-eB.*sin(alphaAB)+LB.*cos(q2).*sin(alphaAB)))./lB-((dz+LB.*dq2.*cos(q2)).*(dx-LB.*dq2.*sin(q2).*cos(alphaAB-pi./2.0)))./lB+((dx-LB.*dq2.*sin(alphaAB).*sin(q2)).*(dz+LB.*dq2.*sin(pi./2.0).*cos(q2)))./lB+((z+LB.*sin(q2)).*(-ddx+LB.*dq2.^2.*cos(q2).*cos(alphaAB-pi./2.0)+LB.*ddq2.*sin(q2).*cos(alphaAB-pi./2.0)))./lB))./(lB.*2.0)).*(x+aB.*sin(alphaAB)-eB.*sin(alphaAB)+LB.*cos(q2).*sin(alphaAB)).*2.0+1.0./lC.^2.*((IlCxy.*(((dz+LC.*dq3.*cos(q3)).*(dy+LC.*dq3.*sin(alphaAC-pi./2.0).*sin(q3)))./lC-((dy-LC.*dq3.*cos(alphaAC).*sin(q3)).*(dz+LC.*dq3.*sin(pi./2.0).*cos(q3)))./lC+((z+LC.*sin(q3)).*(ddy+LC.*dq3.^2.*sin(alphaAC-pi./2.0).*cos(q3)+LC.*ddq3.*sin(alphaAC-pi./2.0).*sin(q3)))./lC-((ddz+LC.*ddq3.*sin(pi./2.0).*cos(q3)-LC.*dq3.^2.*sin(pi./2.0).*sin(q3)).*(y+aC.*cos(alphaAC)-eC.*cos(alphaAC)+LC.*cos(alphaAC).*cos(q3)))./lC))./(lC.*2.0)-(IlCyz.*(-((dy-LC.*dq3.*cos(alphaAC).*sin(q3)).*(dx-LC.*dq3.*sin(q3).*cos(alphaAC-pi./2.0)))./lC+((dx-LC.*dq3.*sin(alphaAC).*sin(q3)).*(dy+LC.*dq3.*sin(alphaAC-pi./2.0).*sin(q3)))./lC+((ddy+LC.*dq3.^2.*sin(alphaAC-pi./2.0).*cos(q3)+LC.*ddq3.*sin(alphaAC-pi./2.0).*sin(q3)).*(x+aC.*sin(alphaAC)-eC.*sin(alphaAC)+LC.*cos(q3).*sin(alphaAC)))./lC+((-ddx+LC.*dq3.^2.*cos(q3).*cos(alphaAC-pi./2.0)+LC.*ddq3.*sin(q3).*cos(alphaAC-pi./2.0)).*(y+aC.*cos(alphaAC)-eC.*cos(alphaAC)+LC.*cos(alphaAC).*cos(q3)))./lC))./(lC.*2.0)+(IlCyy.*(((ddz+LC.*ddq3.*sin(pi./2.0).*cos(q3)-LC.*dq3.^2.*sin(pi./2.0).*sin(q3)).*(x+aC.*sin(alphaAC)-eC.*sin(alphaAC)+LC.*cos(q3).*sin(alphaAC)))./lC-((dz+LC.*dq3.*cos(q3)).*(dx-LC.*dq3.*sin(q3).*cos(alphaAC-pi./2.0)))./lC+((dx-LC.*dq3.*sin(alphaAC).*sin(q3)).*(dz+LC.*dq3.*sin(pi./2.0).*cos(q3)))./lC+((z+LC.*sin(q3)).*(-ddx+LC.*dq3.^2.*cos(q3).*cos(alphaAC-pi./2.0)+LC.*ddq3.*sin(q3).*cos(alphaAC-pi./2.0)))./lC))./(lC.*2.0)).*(x+aC.*sin(alphaAC)-eC.*sin(alphaAC)+LC.*cos(q3).*sin(alphaAC)).*2.0-(((IlAxx.*1.0./lA.^2.*(y+aA.*cos(alphaAA)-eA.*cos(alphaAA)+LA.*cos(alphaAA).*cos(q1)))./2.0-(IlAxy.*1.0./lA.^2.*(x+aA.*sin(alphaAA)-eA.*sin(alphaAA)+LA.*cos(q1).*sin(alphaAA)))./2.0).*(((dz+LA.*dq1.*cos(q1)).*(dy+LA.*dq1.*sin(alphaAA-pi./2.0).*sin(q1)))./lA-((dy-LA.*dq1.*cos(alphaAA).*sin(q1)).*(dz+LA.*dq1.*sin(pi./2.0).*cos(q1)))./lA+((z+LA.*sin(q1)).*(ddy+LA.*dq1.^2.*sin(alphaAA-pi./2.0).*cos(q1)+LA.*ddq1.*sin(alphaAA-pi./2.0).*sin(q1)))./lA-((ddz+LA.*ddq1.*sin(pi./2.0).*cos(q1)-LA.*dq1.^2.*sin(pi./2.0).*sin(q1)).*(y+aA.*cos(alphaAA)-eA.*cos(alphaAA)+LA.*cos(alphaAA).*cos(q1)))./lA).*2.0)./lA-(((IlBxx.*1.0./lB.^2.*(y+aB.*cos(alphaAB)-eB.*cos(alphaAB)+LB.*cos(alphaAB).*cos(q2)))./2.0-(IlBxy.*1.0./lB.^2.*(x+aB.*sin(alphaAB)-eB.*sin(alphaAB)+LB.*cos(q2).*sin(alphaAB)))./2.0).*(((dz+LB.*dq2.*cos(q2)).*(dy+LB.*dq2.*sin(alphaAB-pi./2.0).*sin(q2)))./lB-((dy-LB.*dq2.*cos(alphaAB).*sin(q2)).*(dz+LB.*dq2.*sin(pi./2.0).*cos(q2)))./lB+((z+LB.*sin(q2)).*(ddy+LB.*dq2.^2.*sin(alphaAB-pi./2.0).*cos(q2)+LB.*ddq2.*sin(alphaAB-pi./2.0).*sin(q2)))./lB-((ddz+LB.*ddq2.*sin(pi./2.0).*cos(q2)-LB.*dq2.^2.*sin(pi./2.0).*sin(q2)).*(y+aB.*cos(alphaAB)-eB.*cos(alphaAB)+LB.*cos(alphaAB).*cos(q2)))./lB).*2.0)./lB-(((IlCxx.*1.0./lC.^2.*(y+aC.*cos(alphaAC)-eC.*cos(alphaAC)+LC.*cos(alphaAC).*cos(q3)))./2.0-(IlCxy.*1.0./lC.^2.*(x+aC.*sin(alphaAC)-eC.*sin(alphaAC)+LC.*cos(q3).*sin(alphaAC)))./2.0).*(((dz+LC.*dq3.*cos(q3)).*(dy+LC.*dq3.*sin(alphaAC-pi./2.0).*sin(q3)))./lC-((dy-LC.*dq3.*cos(alphaAC).*sin(q3)).*(dz+LC.*dq3.*sin(pi./2.0).*cos(q3)))./lC+((z+LC.*sin(q3)).*(ddy+LC.*dq3.^2.*sin(alphaAC-pi./2.0).*cos(q3)+LC.*ddq3.*sin(alphaAC-pi./2.0).*sin(q3)))./lC-((ddz+LC.*ddq3.*sin(pi./2.0).*cos(q3)-LC.*dq3.^2.*sin(pi./2.0).*sin(q3)).*(y+aC.*cos(alphaAC)-eC.*cos(alphaAC)+LC.*cos(alphaAC).*cos(q3)))./lC).*2.0)./lC];
